simulink model "COMPONENT_MDL_Lag_QUAD_and_PEND_with_Ab"  (R2020b)
(part 8 of 12)

_Theta_pend))./2.0).*2.0+THE_Theta_D.*cos(THE_Psi).*sin(THE_Theta).*((Lz_pend.*THE_Psi_pend_D.*cos(THE_Theta_pend).*sin(THE_Psi_pend))./2.0+(Lz_pend.*THE_Theta_pend_D.*cos(THE_Psi_pend).*sin(THE_Theta_pend))./2.0).*2.0+Lz_pend.*THE_Psi_D.*cos(THE_Psi).*cos(THE_Theta).*(-THE_Psi_pend_D.*cos(THE_Phi_pend).*cos(THE_Psi_pend)+THE_Phi_pend_D.*sin(THE_Phi_pend).*sin(THE_Psi_pend)-THE_Psi_pend_D.*sin(THE_Phi_pend).*sin(THE_Psi_pend).*sin(THE_Theta_pend)+THE_Phi_pend_D.*cos(THE_Phi_pend).*cos(THE_Psi_pend).*sin(THE_Theta_pend)+THE_Theta_pend_D.*cos(THE_Psi_pend).*cos(THE_Theta_pend).*sin(THE_Phi_pend))-Lz_pend.*THE_Theta_D.*sin(THE_Psi).*sin(THE_Theta).*(-THE_Psi_pend_D.*cos(THE_Phi_pend).*cos(THE_Psi_pend)+THE_Phi_pend_D.*sin(THE_Phi_pend).*sin(THE_Psi_pend)-THE_Psi_pend_D.*sin(THE_Phi_pend).*sin(THE_Psi_pend).*sin(THE_Theta_pend)+THE_Phi_pend_D.*cos(THE_Phi_pend).*cos(THE_Psi_pend).*sin(THE_Theta_pend)+THE_Theta_pend_D.*cos(THE_Psi_pend).*cos(THE_Theta_pend).*sin(THE_Phi_pend))+THE_Psi_D.*THE_Theta_D.*sin(THE_Psi).*sin(THE_Theta).*(Tv_Z_pend+(Lz_pend.*cos(THE_Psi_pend).*cos(THE_Theta_pend))./2.0).*2.0+(Lz_pend.*THE_Psi_D.^2.*cos(THE_Theta).*sin(THE_Psi).*(cos(THE_Phi_pend).*sin(THE_Psi_pend)-cos(THE_Psi_pend).*sin(THE_Phi_pend).*sin(THE_Theta_pend)))./2.0+(Lz_pend.*THE_Theta_D.^2.*cos(THE_Theta).*sin(THE_Psi).*(cos(THE_Phi_pend).*sin(THE_Psi_pend)-cos(THE_Psi_pend).*sin(THE_Phi_pend).*sin(THE_Theta_pend)))./2.0+Lz_pend.*THE_Psi_D.*THE_Theta_D.*cos(THE_Psi).*sin(THE_Theta).*(cos(THE_Phi_pend).*sin(THE_Psi_pend)-cos(THE_Psi_pend).*sin(THE_Phi_pend).*sin(THE_Theta_pend)))+m_pend.*((Lz_pend.*cos(THE_Theta).*(sin(THE_Phi_pend).*sin(THE_Psi_pend)+cos(THE_Phi_pend).*cos(THE_Psi_pend).*sin(THE_Theta_pend)))./2.0+cos(THE_Psi).*sin(THE_Theta).*(Tv_Z_pend+(Lz_pend.*cos(THE_Psi_pend).*cos(THE_Theta_pend))./2.0)-(Lz_pend.*sin(THE_Psi).*sin(THE_Theta).*(cos(THE_Phi_pend).*sin(THE_Psi_pend)-cos(THE_Psi_pend).*sin(THE_Phi_pend).*sin(THE_Theta_pend)))./2.0).*((Lz_pend.*sin(THE_Theta).*(THE_Phi_pend_D.^2.*sin(THE_Phi_pend).*sin(THE_Psi_pend)+THE_Psi_pend_D.^2.*sin(THE_Phi_pend).*sin(THE_Psi_pend)+THE_Phi_pend_D.^2.*cos(THE_Phi_pend).*cos(THE_Psi_pend).*sin(THE_Theta_pend)+THE_Psi_pend_D.^2.*cos(THE_Phi_pend).*cos(THE_Psi_pend).*sin(THE_Theta_pend)+THE_Theta_pend_D.^2.*cos(THE_Phi_pend).*cos(THE_Psi_pend).*sin(THE_Theta_pend)-THE_Phi_pend_D.*THE_Psi_pend_D.*cos(THE_Phi_pend).*cos(THE_Psi_pend).*2.0+THE_Phi_pend_D.*THE_Theta_pend_D.*cos(THE_Psi_pend).*cos(THE_Theta_pend).*sin(THE_Phi_pend).*2.0+THE_Psi_pend_D.*THE_Theta_pend_D.*cos(THE_Phi_pend).*cos(THE_Theta_pend).*sin(THE_Psi_pend).*2.0-THE_Phi_pend_D.*THE_Psi_pend_D.*sin(THE_Phi_pend).*sin(THE_Psi_pend).*sin(THE_Theta_pend).*2.0))./4.0-(cos(THE_Psi).*cos(THE_Theta).*((Lz_pend.*THE_Psi_pend_D.^2.*cos(THE_Psi_pend).*cos(THE_Theta_pend))./2.0+(Lz_pend.*THE_Theta_pend_D.^2.*cos(THE_Psi_pend).*cos(THE_Theta_pend))./2.0-Lz_pend.*THE_Psi_pend_D.*THE_Theta_pend_D.*sin(THE_Psi_pend).*sin(THE_Theta_pend)))./2.0+(Lz_pend.*THE_Theta_D.^2.*sin(THE_Theta).*(sin(THE_Phi_pend).*sin(THE_Psi_pend)+cos(THE_Phi_pend).*cos(THE_Psi_pend).*sin(THE_Theta_pend)))./4.0-(Lz_pend.*cos(THE_Theta).*sin(THE_Psi).*(-THE_Phi_pend_D.^2.*cos(THE_Phi_pend).*sin(THE_Psi_pend)-THE_Psi_pend_D.^2.*cos(THE_Phi_pend).*sin(THE_Psi_pend)+THE_Phi_pend_D.^2.*cos(THE_Psi_pend).*sin(THE_Phi_pend).*sin(THE_Theta_pend)+THE_Psi_pend_D.^2.*cos(THE_Psi_pend).*sin(THE_Phi_pend).*sin(THE_Theta_pend)+THE_Theta_pend_D.^2.*cos(THE_Psi_pend).*sin(THE_Phi_pend).*sin(THE_Theta_pend)-THE_Phi_pend_D.*THE_Psi_pend_D.*cos(THE_Psi_pend).*sin(THE_Phi_pend).*2.0-THE_Phi_pend_D.*THE_Theta_pend_D.*cos(THE_Phi_pend).*cos(THE_Psi_pend).*cos(THE_Theta_pend).*2.0+THE_Phi_pend_D.*THE_Psi_pend_D.*cos(THE_Phi_pend).*sin(THE_Psi_pend).*sin(THE_Theta_pend).*2.0+THE_Psi_pend_D.*THE_Theta_pend_D.*cos(THE_Theta_pend).*sin(THE_Phi_pend).*sin(THE_Psi_pend).*2.0))./4.0-(Lz_pend.*THE_Theta_D.*cos(THE_Theta).*(THE_Phi_pend_D.*cos(THE_Phi_pend).*sin(THE_Psi_pend)+THE_Psi_pend_D.*cos(THE_Psi_pend).*sin(THE_Phi_pend)+THE_Theta_pend_D.*cos(THE_Phi_pend).*cos(THE_Psi_pend).*cos(THE_Theta_pend)-THE_Phi_pend_D.*cos(THE_Psi_pend).*sin(THE_Phi_pend).*sin(THE_Theta_pend)-THE_Psi_pend_D.*cos(THE_Phi_pend).*sin(THE_Psi_pend).*sin(THE_Theta_pend)))./2.0-(THE_Psi_D.^2.*cos(THE_Psi).*cos(THE_Theta).*(Tv_Z_pend+(Lz_pend.*cos(THE_Psi_pend).*cos(THE_Theta_pend))./2.0))./2.0-(THE_Theta_D.^2.*cos(THE_Psi).*cos(THE_Theta).*(Tv_Z_pend+(Lz_pend.*cos(THE_Psi_pend).*cos(THE_Theta_pend))./2.0))./2.0+THE_Psi_D.*cos(THE_Theta).*sin(THE_Psi).*((Lz_pend.*THE_Psi_pend_D.*cos(THE_Theta_pend).*sin(THE_Psi_pend))./2.0+(Lz_pend.*THE_Theta_pend_D.*cos(THE_Psi_pend).*sin(THE_Theta_pend))./2.0)+THE_Theta_D.*cos(THE_Psi).*sin(THE_Theta).*((Lz_pend.*THE_Psi_pend_D.*cos(THE_Theta_pend).*sin(THE_Psi_pend))./2.0+(Lz_pend.*THE_Theta_pend_D.*cos(THE_Psi_pend).*sin(THE_Theta_pend))./2.0)+(Lz_pend.*THE_Psi_D.*cos(THE_Psi).*cos(THE_Theta).*(-THE_Psi_pend_D.*cos(THE_Phi_pend).*cos(THE_Psi_pend)+THE_Phi_pend_D.*sin(THE_Phi_pend).*sin(THE_Psi_pend)-THE_Psi_pend_D.*sin(THE_Phi_pend).*sin(THE_Psi_pend).*sin(THE_Theta_pend)+THE_Phi_pend_D.*cos(THE_Phi_pend).*cos(THE_Psi_pend).*sin(THE_Theta_pend)+THE_Theta_pend_D.*cos(THE_Psi_pend).*cos(THE_Theta_pend).*sin(THE_Phi_pend)))./2.0-(Lz_pend.*THE_Theta_D.*sin(THE_Psi).*sin(THE_Theta).*(-THE_Psi_pend_D.*cos(THE_Phi_pend).*cos(THE_Psi_pend)+THE_Phi_pend_D.*sin(THE_Phi_pend).*sin(THE_Psi_pend)-THE_Psi_pend_D.*sin(THE_Phi_pend).*sin(THE_Psi_pend).*sin(THE_Theta_pend)+THE_Phi_pend_D.*cos(THE_Phi_pend).*cos(THE_Psi_pend).*sin(THE_Theta_pend)+THE_Theta_pend_D.*cos(THE_Psi_pend).*cos(THE_Theta_pend).*sin(THE_Phi_pend)))./2.0+THE_Psi_D.*THE_Theta_D.*sin(THE_Psi).*sin(THE_Theta).*(Tv_Z_pend+(Lz_pend.*cos(THE_Psi_pend).*cos(THE_Theta_pend))./2.0)+(Lz_pend.*THE_Psi_D.^2.*cos(THE_Theta).*sin(THE_Psi).*(cos(THE_Phi_pend).*sin(THE_Psi_pend)-cos(THE_Psi_pend).*sin(THE_Phi_pend).*sin(THE_Theta_pend)))./4.0+(Lz_pend.*THE_Theta_D.^2.*cos(THE_Theta).*sin(THE_Psi).*(cos(THE_Phi_pend).*sin(THE_Psi_pend)-cos(THE_Psi_pend).*sin(THE_Phi_pend).*sin(THE_Theta_pend)))./4.0+(Lz_pend.*THE_Psi_D.*THE_Theta_D.*cos(THE_Psi).*sin(THE_Theta).*(cos(THE_Phi_pend).*sin(THE_Psi_pend)-cos(THE_Psi_pend).*sin(THE_Phi_pend).*sin(THE_Theta_pend)))./2.0)-mprop.*(THE_Y_D-(cg_to_mot_L.*(THE_Theta_D.*sin(THE_Psi)-THE_Phi_D.*cos(THE_Psi).*cos(THE_Theta))+cg_to_mot_H.*(THE_Psi_D-THE_Phi_D.*sin(THE_Theta))).*(cos(THE_Phi).*cos(THE_Psi)+sin(THE_Phi).*sin(THE_Psi).*sin(THE_Theta))+cg_to_mot_L.*(cos(THE_Phi).*sin(THE_Psi)-cos(THE_Psi).*sin(THE_Phi).*sin(THE_Theta)).*(THE_Theta_D.*cos(THE_Psi)+THE_Phi_D.*cos(THE_Theta).*sin(THE_Psi))+cg_to_mot_H.*cos(THE_Theta).*sin(THE_Phi).*(THE_Theta_D.*cos(THE_Psi)+THE_Phi_D.*cos(THE_Theta).*sin(THE_Psi))).*((THE_Phi_D.*cg_to_mot_H.*cos(THE_Theta)-THE_Phi_D.*cg_to_mot_L.*cos(THE_Psi).*sin(THE_Theta)).*(cos(THE_Phi).*cos(THE_Psi)+sin(THE_Phi).*sin(THE_Psi).*sin(THE_Theta)).*(-1.0./2.0)+(cg_to_mot_H.*sin(THE_Phi).*sin(THE_Theta).*(THE_Theta_D.*cos(THE_Psi)+THE_Phi_D.*cos(THE_Theta).*sin(THE_Psi)))./2.0+(cos(THE_Theta).*sin(THE_Phi).*sin(THE_Psi).*(cg_to_mot_L.*(THE_Theta_D.*sin(THE_Psi)-THE_Phi_D.*cos(THE_Psi).*cos(THE_Theta))+cg_to_mot_H.*(THE_Psi_D-THE_Phi_D.*sin(THE_Theta))))./2.0+(THE_Phi_D.*cg_to_mot_L.*sin(THE_Psi).*sin(THE_Theta).*(cos(THE_Phi).*sin(THE_Psi)-cos(THE_Psi).*sin(THE_Phi).*sin(THE_Theta)))./2.0+(cg_to_mot_L.*cos(THE_Psi).*cos(THE_Theta).*sin(THE_Phi).*(THE_Theta_D.*cos(THE_Psi)+THE_Phi_D.*cos(THE_Theta).*sin(THE_Psi)))./2.0+(THE_Phi_D.*cg_to_mot_H.*cos(THE_Theta).*sin(THE_Phi).*sin(THE_Psi).*sin(THE_Theta))./2.0)+mprop.*(THE_Y_D+(cg_to_mot_L.*(THE_Theta_D.*sin(THE_Psi)-THE_Phi_D.*cos(THE_Psi).*cos(THE_Theta))-cg_to_mot_H.*(THE_Psi_D-THE_Phi_D.*sin(THE_Theta))).*(cos(THE_Phi).*cos(THE_Psi)+sin(THE_Phi).*sin(THE_Psi).*sin(THE_Theta))-cg_to_mot_L.*(cos(THE_Phi).*sin(THE_Psi)-cos(THE_Psi).*sin(THE_Phi).*sin(THE_Theta)).*(THE_Theta_D.*cos(THE_Psi)+THE_Phi_D.*cos(THE_Theta).*sin(THE_Psi))+cg_to_mot_H.*cos(THE_Theta).*sin(THE_Phi).*(THE_Theta_D.*cos(THE_Psi)+THE_Phi_D.*cos(THE_Theta).*sin(THE_Psi))).*(((THE_Phi_D.*cg_to_mot_H.*cos(THE_Theta)+THE_Phi_D.*cg_to_mot_L.*cos(THE_Psi).*sin(THE_Theta)).*(cos(THE_Phi).*cos(THE_Psi)+sin(THE_Phi).*sin(THE_Psi).*sin(THE_Theta)))./2.0-(cg_to_mot_H.*sin(THE_Phi).*sin(THE_Theta).*(THE_Theta_D.*cos(THE_Psi)+THE_Phi_D.*cos(THE_Theta).*sin(THE_Psi)))./2.0+(cos(THE_Theta).*sin(THE_Phi).*sin(THE_Psi).*(cg_to_mot_L.*(THE_Theta_D.*sin(THE_Psi)-THE_Phi_D.*cos(THE_Psi).*cos(THE_Theta))-cg_to_mot_H.*(THE_Psi_D-THE_Phi_D.*sin(THE_Theta))))./2.0+(THE_Phi_D.*cg_to_mot_L.*sin(THE_Psi).*sin(THE_Theta).*(cos(THE_Phi).*sin(THE_Psi)-cos(THE_Psi).*sin(THE_Phi).*sin(THE_Theta)))./2.0+(cg_to_mot_L.*cos(THE_Psi).*cos(THE_Theta).*sin(THE_Phi).*(THE_Theta_D.*cos(THE_Psi)+THE_Phi_D.*cos(THE_Theta).*sin(THE_Psi)))./2.0-(THE_Phi_D.*cg_to_mot_H.*cos(THE_Theta).*sin(THE_Phi).*sin(THE_Psi).*sin(THE_Theta))./2.0)-mprop.*(THE_X_D./2.0+((cg_to_mot_L.*(THE_Theta_D.*sin(THE_Psi)-THE_Phi_D.*cos(THE_Psi).*cos(THE_Theta))+cg_to_mot_H.*(THE_Psi_D-THE_Phi_D.*sin(THE_Theta))).*(cos(THE_Psi).*sin(THE_Phi)-cos(THE_Phi).*sin(THE_Psi).*sin(THE_Theta)))./2.0-(cg_to_mot_L.*(sin(THE_Phi).*sin(THE_Psi)+cos(THE_Phi).*cos(THE_Psi).*sin(THE_Theta)).*(THE_Theta_D.*cos(THE_Psi)+THE_Phi_D.*cos(THE_Theta).*sin(THE_Psi)))./2.0+(cg_to_mot_H.*cos(THE_Phi).*cos(THE_Theta).*(THE_Theta_D.*cos(THE_Psi)+THE_Phi_D.*cos(THE_Theta).*sin(THE_Psi)))./2.0).*((THE_Phi_D.*cg_to_mot_H.*cos(THE_Theta)-THE_Phi_D.*cg_to_mot_L.*cos(THE_Psi).*sin(THE_Theta)).*(cos(THE_Psi).*sin(THE_Phi)-cos(THE_Phi).*sin(THE_Psi).*sin(THE_Theta))+cg_to_mot_H.*cos(THE_Phi).*sin(THE_Theta).*(THE_Theta_D.*cos(THE_Psi)+THE_Phi_D.*cos(THE_Theta).*sin(THE_Psi))+cos(THE_Phi).*cos(THE_Theta).*sin(THE_Psi).*(cg_to_mot_L.*(THE_Theta_D.*sin(THE_Psi)-THE_Phi_D.*cos(THE_Psi).*cos(THE_Theta))+cg_to_mot_H.*(THE_Psi_D-THE_Phi_D.*sin(THE_Theta)))-THE_Phi_D.*cg_to_mot_L.*sin(THE_Psi).*sin(THE_Theta).*(sin(THE_Phi).*sin(THE_Psi)+cos(THE_Phi).*cos(THE_Psi).*sin(THE_Theta))+cg_to_mot_L.*cos(THE_Phi).*cos(THE_Psi).*cos(THE_Theta).*(THE_Theta_D.*cos(THE_Psi)+THE_Phi_D.*cos(THE_Theta).*sin(THE_Psi))+THE_Phi_D.*cg_to_mot_H.*cos(THE_Phi).*cos(THE_Theta).*sin(THE_Psi).*sin(THE_Theta))-mprop.*(THE_X_D./2.0-((cg_to_mot_L.*(THE_Theta_D.*sin(THE_Psi)-THE_Phi_D.*cos(THE_Psi).*cos(THE_Theta))-cg_to_mot_H.*(THE_Psi_D-THE_Phi_D.*sin(THE_Theta))).*(cos(THE_Psi).*sin(THE_Phi)-cos(THE_Phi).*sin(THE_Psi).*sin(THE_Theta)))./2.0+(cg_to_mot_L.*(sin(THE_Phi).*sin(THE_Psi)+cos(THE_Phi).*cos(THE_Psi).*sin(THE_Theta)).*(THE_Theta_D.*cos(THE_Psi)+THE_Phi_D.*cos(THE_Theta).*sin(THE_Psi)))./2.0+(cg_to_mot_H.*cos(THE_Phi).*cos(THE_Theta).*(THE_Theta_D.*cos(THE_Psi)+THE_Phi_D.*cos(THE_Theta).*sin(THE_Psi)))./2.0).*((THE_Phi_D.*cg_to_mot_H.*cos(THE_Theta)+THE_Phi_D.*cg_to_mot_L.*cos(THE_Psi).*sin(THE_Theta)).*(cos(THE_Psi).*sin(THE_Phi)-cos(THE_Phi).*sin(THE_Psi).*sin(THE_Theta))+cg_to_mot_H.*cos(THE_Phi).*sin(THE_Theta).*(THE_Theta_D.*cos(THE_Psi)+THE_Phi_D.*cos(THE_Theta).*sin(THE_Psi))-cos(THE_Phi).*cos(THE_Theta).*sin(THE_Psi).*(cg_to_mot_L.*(THE_Theta_D.*sin(THE_Psi)-THE_Phi_D.*cos(THE_Psi).*cos(THE_Theta))-cg_to_mot_H.*(THE_Psi_D-THE_Phi_D.*sin(THE_Theta)))+THE_Phi_D.*cg_to_mot_L.*sin(THE_Psi).*sin(THE_Theta).*(sin(THE_Phi).*sin(THE_Psi)+cos(THE_Phi).*cos(THE_Psi).*sin(THE_Theta))-cg_to_mot_L.*cos(THE_Phi).*cos(THE_Psi).*cos(THE_Theta).*(THE_Theta_D.*cos(THE_Psi)+THE_Phi_D.*cos(THE_Theta).*sin(THE_Psi))+THE_Phi_D.*cg_to_mot_H.*cos(THE_Phi).*cos(THE_Theta).*sin(THE_Psi).*sin(THE_Theta))+mprop.*(cg_to_mot_L.*cos(THE_Psi).*(sin(THE_Phi).*sin(THE_Psi)+cos(THE_Phi).*cos(THE_Psi).*sin(THE_Theta)).*(-1.0./2.0)+(cg_to_mot_L.*sin(THE_Psi).*(cos(THE_Psi).*sin(THE_Phi)-cos(THE_Phi).*sin(THE_Psi).*sin(THE_Theta)))./2.0+(cg_to_mot_H.*cos(THE_Phi).*cos(THE_Psi).*cos(THE_Theta))./2.0).*((cg_to_mot_L.*(THE_Theta_D.*sin(THE_Psi)-THE_Phi_D.*cos(THE_Psi).*cos(THE_Theta))+cg_to_mot_H.*(THE_Psi_D-THE_Phi_D.*sin(THE_Theta))).*(-THE_Phi_D.*cos(THE_Phi).*cos(THE_Psi)+THE_Psi_D.*sin(THE_Phi).*sin(THE_Psi)-THE_Phi_D.*sin(THE_Phi).*sin(THE_Psi).*sin(THE_Theta)+THE_Psi_D.*cos(THE_Phi).*cos(THE_Psi).*sin(THE_Theta)+THE_Theta_D.*cos(THE_Phi).*cos(THE_Theta).*sin(THE_Psi))-(cg_to_mot_L.*(THE_Psi_D.*THE_Theta_D.*cos(THE_Psi)+THE_Phi_D.*THE_Psi_D.*cos(THE_Theta).*sin(THE_Psi)+THE_Phi_D.*THE_Theta_D.*cos(THE_Psi).*sin(THE_Theta))-THE_Phi_D.*THE_Theta_D.*cg_to_mot_H.*cos(THE_Theta)).*(cos(THE_Psi).*sin(THE_Phi)-cos(THE_Phi).*sin(THE_Psi).*sin(THE_Theta))+cg_to_mot_L.*(THE_Theta_D.*cos(THE_Psi)+THE_Phi_D.*cos(THE_Theta).*sin(THE_Psi)).*(THE_Phi_D.*cos(THE_Phi).*sin(THE_Psi)+THE_Psi_D.*cos(THE_Psi).*sin(THE_Phi)+THE_Theta_D.*cos(THE_Phi).*cos(THE_Psi).*cos(THE_Theta)-THE_Phi_D.*cos(THE_Psi).*sin(THE_Phi).*sin(THE_Theta)-THE_Psi_D.*cos(THE_Phi).*sin(THE_Psi).*sin(THE_Theta))-cg_to_mot_L.*(sin(THE_Phi).*sin(THE_Psi)+cos(THE_Phi).*cos(THE_Psi).*sin(THE_Theta)).*(THE_Psi_D.*THE_Theta_D.*sin(THE_Psi)-THE_Phi_D.*THE_Psi_D.*cos(THE_Psi).*cos(THE_Theta)+THE_Phi_D.*THE_Theta_D.*sin(THE_Psi).*sin(THE_Theta))+cg_to_mot_H.*cos(THE_Phi).*cos(THE_Theta).*(THE_Psi_D.*THE_Theta_D.*sin(THE_Psi)-THE_Phi_D.*THE_Psi_D.*cos(THE_Psi).*cos(THE_Theta)+THE_Phi_D.*THE_Theta_D.*sin(THE_Psi).*sin(THE_Theta))+THE_Phi_D.*cg_to_mot_H.*cos(THE_Theta).*sin(THE_Phi).*(THE_Theta_D.*cos(THE_Psi)+THE_Phi_D.*cos(THE_Theta).*sin(THE_Psi))+THE_Theta_D.*cg_to_mot_H.*cos(THE_Phi).*sin(THE_Theta).*(THE_Theta_D.*cos(THE_Psi)+THE_Phi_D.*cos(THE_Theta).*sin(THE_Psi)))+mprop.*((cg_to_mot_L.*cos(THE_Psi).*(sin(THE_Phi).*sin(THE_Psi)+cos(THE_Phi).*cos(THE_Psi).*sin(THE_Theta)))./2.0-(cg_to_mot_L.*sin(THE_Psi).*(cos(THE_Psi).*sin(THE_Phi)-cos(THE_Phi).*sin(THE_Psi).*sin(THE_Theta)))./2.0+(cg_to_mot_H.*cos(THE_Phi).*cos(THE_Psi).*cos(THE_Theta))./2.0).*(-(cg_to_mot_L.*(THE_Theta_D.*sin(THE_Psi)-THE_Phi_D.*cos(THE_Psi).*cos(THE_Theta))-cg_to_mot_H.*(THE_Psi_D-THE_Phi_D.*sin(THE_Theta))).*(-THE_Phi_D.*cos(THE_Phi).*cos(THE_Psi)+THE_Psi_D.*sin(THE_Phi).*sin(THE_Psi)-THE_Phi_D.*sin(THE_Phi).*sin(THE_Psi).*sin(THE_Theta)+THE_Psi_D.*cos(THE_Phi).*cos(THE_Psi).*sin(THE_Theta)+THE_Theta_D.*cos(THE_Phi).*cos(THE_Theta).*sin(THE_Psi))+(cg_to_mot_L.*(THE_Psi_D.*THE_Theta_D.*cos(THE_Psi)+THE_Phi_D.*THE_Psi_D.*cos(THE_Theta).*sin(THE_Psi)+THE_Phi_D.*THE_Theta_D.*cos(THE_Psi).*sin(THE_Theta))+THE_Phi_D.*THE_Theta_D.*cg_to_mot_H.*cos(THE_Theta)).*(cos(THE_Psi).*sin(THE_Phi)-cos(THE_Phi).*sin(THE_Psi).*sin(THE_Theta))-cg_to_mot_L.*(THE_Theta_D.*cos(THE_Psi)+THE_Phi_D.*cos(THE_Theta).*sin(THE_Psi)).*(THE_Phi_D.*cos(THE_Phi).*sin(THE_Psi)+THE_Psi_D.*cos(THE_Psi).*sin(THE_Phi)+THE_Theta_D.*cos(THE_Phi).*cos(THE_Psi).*cos(THE_Theta)-THE_Phi_D.*cos(THE_Psi).*sin(THE_Phi).*sin(THE_Theta)-THE_Psi_D.*cos(THE_Phi).*sin(THE_Psi).*sin(THE_Theta))+cg_to_mot_L.*(sin(THE_Phi).*sin(THE_Psi)+cos(THE_Phi).*cos(THE_Psi).*sin(THE_Theta)).*(THE_Psi_D.*THE_Theta_D.*sin(THE_Psi)-THE_Phi_D.*THE_Psi_D.*cos(THE_Psi).*cos(THE_Theta)+THE_Phi_D.*THE_Theta_D.*sin(THE_Psi).*sin(THE_Theta))+cg_to_mot_H.*cos(THE_Phi).*cos(THE_Theta).*(THE_Psi_D.*THE_Theta_D.*sin(THE_Psi)-THE_Phi_D.*THE_Psi_D.*cos(THE_Psi).*cos(THE_Theta)+THE_Phi_D.*THE_Theta_D.*sin(THE_Psi).*sin(THE_Theta))+THE_Phi_D.*cg_to_mot_H.*cos(THE_Theta).*sin(THE_Phi).*(THE_Theta_D.*cos(THE_Psi)+THE_Phi_D.*cos(THE_Theta).*sin(THE_Psi))+THE_Theta_D.*cg_to_mot_H.*cos(THE_Phi).*sin(THE_Theta).*(THE_Theta_D.*cos(THE_Psi)+THE_Phi_D.*cos(THE_Theta).*sin(THE_Psi)))+mprop.*(cg_to_mot_L.*cos(THE_Psi).*(sin(THE_Phi).*sin(THE_Psi)+cos(THE_Phi).*cos(THE_Psi).*sin(THE_Theta))-cg_to_mot_L.*sin(THE_Psi).*(cos(THE_Psi).*sin(THE_Phi)-cos(THE_Phi).*sin(THE_Psi).*sin(THE_Theta))+cg_to_mot_H.*cos(THE_Phi).*cos(THE_Psi).*cos(THE_Theta)).*((cg_to_mot_L.*(THE_Theta_D.*sin(THE_Psi)-THE_Phi_D.*cos(THE_Psi).*cos(THE_Theta))-cg_to_mot_H.*(THE_Psi_D-THE_Phi_D.*sin(THE_Theta))).*(-THE_Phi_D.*cos(THE_Phi).*cos(THE_Psi)+THE_Psi_D.*sin(THE_Phi).*sin(THE_Psi)-THE_Phi_D.*sin(THE_Phi).*sin(THE_Psi).*sin(THE_Theta)+THE_Psi_D.*cos(THE_Phi).*cos(THE_Psi).*sin(THE_Theta)+THE_Theta_D.*cos(THE_Phi).*cos(THE_Theta).*sin(THE_Psi)).*(-1.0./2.0)+((cg_to_mot_L.*(THE_Psi_D.*THE_Theta_D.*cos(THE_Psi)+THE_Phi_D.*THE_Psi_D.*cos(THE_Theta).*sin(THE_Psi)+THE_Phi_D.*THE_Theta_D.*cos(THE_Psi).*sin(THE_Theta))+THE_Phi_D.*THE_Theta_D.*cg_to_mot_H.*cos(THE_Theta)).*(cos(THE_Psi).*sin(THE_Phi)-cos(THE_Phi).*sin(THE_Psi).*sin(THE_Theta)))./2.0-(cg_to_mot_L.*(THE_Theta_D.*cos(THE_Psi)+THE_Phi_D.*cos(THE_Theta).*sin(THE_Psi)).*(THE_Phi_D.*cos(THE_Phi).*sin(THE_Psi)+THE_Psi_D.*cos(THE_Psi).*sin(THE_Phi)+THE_Theta_D.*cos(THE_Phi).*cos(THE_Psi).*cos(THE_Theta)-THE_Phi_D.*cos(THE_Psi).*sin(THE_Phi).*sin(THE_Theta)-THE_Psi_D.*cos(THE_Phi).*sin(THE_Psi).*sin(THE_Theta)))./2.0+(cg_to_mot_L.*(sin(THE_Phi).*sin(THE_Psi)+cos(THE_Phi).*cos(THE_Psi).*sin(THE_Theta)).*(THE_Psi_D.*THE_Theta_D.*sin(THE_Psi)-THE_Phi_D.*THE_Psi_D.*cos(THE_Psi).*cos(THE_Theta)+THE_Phi_D.*THE_Theta_D.*sin(THE_Psi).*sin(THE_Theta)))./2.0+(cg_to_mot_H.*cos(THE_Phi).*cos(THE_Theta).*(THE_Psi_D.*THE_Theta_D.*sin(THE_Psi)-THE_Phi_D.*THE_Psi_D.*cos(THE_Psi).*cos(THE_Theta)+THE_Phi_D.*THE_Theta_D.*sin(THE_Psi).*sin(THE_Theta)))./2.0+(THE_Phi_D.*cg_to_mot_H.*cos(THE_Theta).*sin(THE_Phi).*(THE_Theta_D.*cos(THE_Psi)+THE_Phi_D.*cos(THE_Theta).*sin(THE_Psi)))./2.0+(THE_Theta_D.*cg_to_mot_H.*cos(THE_Phi).*sin(THE_Theta).*(THE_Theta_D.*cos(THE_Psi)+THE_Phi_D.*cos(THE_Theta).*sin(THE_Psi)))./2.0)+mprop.*(-cg_to_mot_L.*cos(THE_Psi).*(sin(THE_Phi).*sin(THE_Psi)+cos(THE_Phi).*cos(THE_Psi).*sin(THE_Theta))+cg_to_mot_L.*sin(THE_Psi).*(cos(THE_Psi).*sin(THE_Phi)-cos(THE_Phi).*sin(THE_Psi).*sin(THE_Theta))+cg_to_mot_H.*cos(THE_Phi).*cos(THE_Psi).*cos(THE_Theta)).*(((cg_to_mot_L.*(THE_Theta_D.*sin(THE_Psi)-THE_Phi_D.*cos(THE_Psi).*cos(THE_Theta))+cg_to_mot_H.*(THE_Psi_D-THE_Phi_D.*sin(THE_Theta))).*(-THE_Phi_D.*cos(THE_Phi).*cos(THE_Psi)+THE_Psi_D.*sin(THE_Phi).*sin(THE_Psi)-THE_Phi_D.*sin(THE_Phi).*sin(THE_Psi).*sin(THE_Theta)+THE_Psi_D.*cos(THE_Phi).*cos(THE_Psi).*sin(THE_Theta)+THE_Theta_D.*cos(THE_Phi).*cos(THE_Theta).*sin(THE_Psi)))./2.0-((cg_to_mot_L.*(THE_Psi_D.*THE_Theta_D.*cos(THE_Psi)+THE_Phi_D.*THE_Psi_D.*cos(THE_Theta).*sin(THE_Psi)+THE_Phi_D.*THE_Theta_D.*cos(THE_Psi).*sin(THE_Theta))-THE_Phi_D.*THE_Theta_D.*cg_to_mot_H.*cos(THE_Theta)).*(cos(THE_Psi).*sin(THE_Phi)-cos(THE_Phi).*sin(THE_Psi).*sin(THE_Theta)))./2.0+(cg_to_mot_L.*(THE_Theta_D.*cos(THE_Psi)+THE_Phi_D.*cos(THE_Theta).*sin(THE_Psi)).*(THE_Phi_D.*cos(THE_Phi).*sin(THE_Psi)+THE_Psi_D.*cos(THE_Psi).*sin(THE_Phi)+THE_Theta_D.*cos(THE_Phi).*cos(THE_Psi).*cos(THE_Theta)-THE_Phi_D.*cos(THE_Psi).*sin(THE_Phi).*sin(THE_Theta)-THE_Psi_D.*cos(THE_Phi).*sin(THE_Psi).*sin(THE_Theta)))./2.0-(cg_to_mot_L.*(sin(THE_Phi).*sin(THE_Psi)+cos(THE_Phi).*cos(THE_Psi).*sin(THE_Theta)).*(THE_Psi_D.*THE_Theta_D.*sin(THE_Psi)-THE_Phi_D.*THE_Psi_D.*cos(THE_Psi).*cos(THE_Theta)+THE_Phi_D.*THE_Theta_D.*sin(THE_Psi).*sin(THE_Theta)))./2.0+(cg_to_mot_H.*cos(THE_Phi).*cos(THE_Theta).*(THE_Psi_D.*THE_Theta_D.*sin(THE_Psi)-THE_Phi_D.*THE_Psi_D.*cos(THE_Psi).*cos(THE_Theta)+THE_Phi_D.*THE_Theta_D.*sin(THE_Psi).*sin(THE_Theta)))./2.0+(THE_Phi_D.*cg_to_mot_H.*cos(THE_Theta).*sin(THE_Phi).*(THE_Theta_D.*cos(THE_Psi)+THE_Phi_D.*cos(THE_Theta).*sin(THE_Psi)))./2.0+(THE_Theta_D.*cg_to_mot_H.*cos(THE_Phi).*sin(THE_Theta).*(THE_Theta_D.*cos(THE_Psi)+THE_Phi_D.*cos(THE_Theta).*sin(THE_Psi)))./2.0)+mprop.*(THE_Y_D-(cg_to_mot_L.*(THE_Theta_D.*sin(THE_Psi)-THE_Phi_D.*cos(THE_Psi).*cos(THE_Theta))+cg_to_mot_H.*(THE_Psi_D-THE_Phi_D.*sin(THE_Theta))).*(cos(THE_Phi).*cos(THE_Psi)+sin(THE_Phi).*sin(THE_Psi).*sin(THE_Theta))+cg_to_mot_L.*(cos(THE_Phi).*sin(THE_Psi)-cos(THE_Psi).*sin(THE_Phi).*sin(THE_Theta)).*(THE_Theta_D.*cos(THE_Psi)+THE_Phi_D.*cos(THE_Theta).*sin(THE_Psi))+cg_to_mot_H.*cos(THE_Theta).*sin(THE_Phi).*(THE_Theta_D.*cos(THE_Psi)+THE_Phi_D.*cos(THE_Theta).*sin(THE_Psi))).*((cg_to_mot_L.*cos(THE_Psi).*(-THE_Psi_D.*cos(THE_Phi).*cos(THE_Psi)+THE_Phi_D.*sin(THE_Phi).*sin(THE_Psi)-THE_Psi_D.*sin(THE_Phi).*sin(THE_Psi).*sin(THE_Theta)+THE_Phi_D.*cos(THE_Phi).*cos(THE_Psi).*sin(THE_Theta)+THE_Theta_D.*cos(THE_Psi).*cos(THE_Theta).*sin(THE_Phi)))./2.0+(cg_to_mot_L.*sin(THE_Psi).*(-THE_Phi_D.*cos(THE_Psi).*sin(THE_Phi)-THE_Psi_D.*cos(THE_Phi).*sin(THE_Psi)+THE_Phi_D.*cos(THE_Phi).*sin(THE_Psi).*sin(THE_Theta)+THE_Psi_D.*cos(THE_Psi).*sin(THE_Phi).*sin(THE_Theta)+THE_Theta_D.*cos(THE_Theta).*sin(THE_Phi).*sin(THE_Psi)))./2.0+(THE_Psi_D.*cg_to_mot_L.*cos(THE_Psi).*(cos(THE_Phi).*cos(THE_Psi)+sin(THE_Phi).*sin(THE_Psi).*sin(THE_Theta)))./2.0+(THE_Psi_D.*cg_to_mot_L.*sin(THE_Psi).*(cos(THE_Phi).*sin(THE_Psi)-cos(THE_Psi).*sin(THE_Phi).*sin(THE_Theta)))./2.0-(THE_Phi_D.*cg_to_mot_H.*cos(THE_Phi).*cos(THE_Psi).*cos(THE_Theta))./2.0+(THE_Psi_D.*cg_to_mot_H.*cos(THE_Theta).*sin(THE_Phi).*sin(THE_Psi))./2.0+(THE_Theta_D.*cg_to_mot_H.*cos(THE_Psi).*sin(THE_Phi).*sin(THE_Theta))./2.0)-mprop.*(THE_Y_D+(cg_to_mot_L.*(THE_Theta_D.*sin(THE_Psi)-THE_Phi_D.*cos(THE_Psi).*cos(THE_Theta))-cg_to_mot_H.*(THE_Psi_D-THE_Phi_D.*sin(THE_Theta))).*(cos(THE_Phi).*cos(THE_Psi)+sin(THE_Phi).*sin(THE_Psi).*sin(THE_Theta))-cg_to_mot_L.*(cos(THE_Phi).*sin(THE_Psi)-cos(THE_Psi).*sin(THE_Phi).*sin(THE_Theta)).*(THE_Theta_D.*cos(THE_Psi)+THE_Phi_D.*cos(THE_Theta).*sin(THE_Psi))+cg_to_mot_H.*cos(THE_Theta).*sin(THE_Phi).*(THE_Theta_D.*cos(THE_Psi)+THE_Phi_D.*cos(THE_Theta).*sin(THE_Psi))).*((cg_to_mot_L.*cos(THE_Psi).*(-THE_Psi_D.*cos(THE_Phi).*cos(THE_Psi)+THE_Phi_D.*sin(THE_Phi).*sin(THE_Psi)-THE_Psi_D.*sin(THE_Phi).*sin(THE_Psi).*sin(THE_Theta)+THE_Phi_D.*cos(THE_Phi).*cos(THE_Psi).*sin(THE_Theta)+THE_Theta_D.*cos(THE_Psi).*cos(THE_Theta).*sin(THE_Phi)))./2.0+(cg_to_mot_L.*sin(THE_Psi).*(-THE_Phi_D.*cos(THE_Psi).*sin(THE_Phi)-THE_Psi_D.*cos(THE_Phi).*sin(THE_Psi)+THE_Phi_D.*cos(THE_Phi).*sin(THE_Psi).*sin(THE_Theta)+THE_Psi_D.*cos(THE_Psi).*sin(THE_Phi).*sin(THE_Theta)+THE_Theta_D.*cos(THE_Theta).*sin(THE_Phi).*sin(THE_Psi)))./2.0+(THE_Psi_D.*cg_to_mot_L.*cos(THE_Psi).*(cos(THE_Phi).*cos(THE_Psi)+sin(THE_Phi).*sin(THE_Psi).*sin(THE_Theta)))./2.0+(THE_Psi_D.*cg_to_mot_L.*sin(THE_Psi).*(cos(THE_Phi).*sin(THE_Psi)-cos(THE_Psi).*sin(THE_Phi).*sin(THE_Theta)))./2.0+(THE_Phi_D.*cg_to_mot_H.*cos(THE_Phi).*cos(THE_Psi).*cos(THE_Theta))./2.0-(THE_Psi_D.*cg_to_mot_H.*cos(THE_Theta).*sin(THE_Phi).*sin(THE_Psi))./2.0-(THE_Theta_D.*cg_to_mot_H.*cos(THE_Psi).*sin(THE_Phi).*sin(THE_Theta))./2.0)-m_pend.*(Ly_pend.^2./1.2e+1+Lz_pend.^2./1.2e+1).*(THE_Psi_pend_D+sin(THE_Theta_pend).*(THE_Theta_D.*sin(THE_Psi)-THE_Phi_D.*cos(THE_Psi).*cos(THE_Theta))-THE_Phi_pend_D.*sin(THE_Theta_pend)+cos(THE_Theta_pend).*sin(THE_Phi_pend).*(THE_Theta_D.*cos(THE_Psi)+THE_Phi_D.*cos(THE_Theta).*sin(THE_Psi))+cos(THE_Phi_pend).*cos(THE_Theta_pend).*(THE_Psi_D-THE_Phi_D.*sin(THE_Theta))).*((THE_Psi_D.*cos(THE_Psi).*sin(THE_Theta_pend))./2.0+(THE_Theta_pend_D.*cos(THE_Theta_pend).*sin(THE_Psi))./2.0+(THE_Phi_pend_D.*cos(THE_Psi).*cos(THE_Phi_pend).*cos(THE_Theta_pend))./2.0-(THE_Psi_D.*cos(THE_Theta_pend).*sin(THE_Psi).*sin(THE_Phi_pend))./2.0-(THE_Theta_pend_D.*cos(THE_Psi).*sin(THE_Phi_pend).*sin(THE_Theta_pend))./2.0)+m_pend.*(Lx_pend.^2./1.2e+1+Ly_pend.^2./1.2e+1).*(cos(THE_Psi).*(-THE_Psi_pend_D.*cos(THE_Phi_pend).*cos(THE_Psi_pend)+THE_Phi_pend_D.*sin(THE_Phi_pend).*sin(THE_Psi_pend)-THE_Psi_pend_D.*sin(THE_Phi_pend).*sin(THE_Psi_pend).*sin(THE_Theta_pend)+THE_Phi_pend_D.*cos(THE_Phi_pend).*cos(THE_Psi_pend).*sin(THE_Theta_pend)+THE_Theta_pend_D.*cos(THE_Psi_pend).*cos(THE_Theta_pend).*sin(THE_Phi_pend))+THE_Psi_D.*sin(THE_Psi).*(cos(THE_Phi_pend).*sin(THE_Psi_pend)-cos(THE_Psi_pend).*sin(THE_Phi_pend).*sin(THE_Theta_pend))-THE_Psi_D.*cos(THE_Psi).*cos(THE_Psi_pend).*cos(THE_Theta_pend)+THE_Psi_pend_D.*cos(THE_Theta_pend).*sin(THE_Psi).*sin(THE_Psi_pend)+THE_Theta_pend_D.*cos(THE_Psi_pend).*sin(THE_Psi).*sin(THE_Theta_pend)).*(((cos(THE_Phi_pend).*sin(THE_Psi_pend)-cos(THE_Psi_pend).*sin(THE_Phi_pend).*sin(THE_Theta_pend)).*(THE_Theta_D.*cos(THE_Psi)+THE_Phi_D.*cos(THE_Theta).*sin(THE_Psi)))./2.0-((THE_Psi_D-THE_Phi_D.*sin(THE_Theta)).*(sin(THE_Phi_pend).*sin(THE_Psi_pend)+cos(THE_Phi_pend).*cos(THE_Psi_pend).*sin(THE_Theta_pend)))./2.0+(THE_Theta_pend_D.*sin(THE_Psi_pend))./2.0-(THE_Phi_pend_D.*cos(THE_Psi_pend).*cos(THE_Theta_pend))./2.0+(cos(THE_Psi_pend).*cos(THE_Theta_pend).*(THE_Theta_D.*sin(THE_Psi)-THE_Phi_D.*cos(THE_Psi).*cos(THE_Theta)))./2.0)+m_pend.*(Lx_pend.^2./1.2e+1+Ly_pend.^2./1.2e+1).*((cos(THE_Psi).*(-THE_Psi_pend_D.*cos(THE_Phi_pend).*cos(THE_Psi_pend)+THE_Phi_pend_D.*sin(THE_Phi_pend).*sin(THE_Psi_pend)-THE_Psi_pend_D.*sin(THE_Phi_pend).*sin(THE_Psi_pend).*sin(THE_Theta_pend)+THE_Phi_pend_D.*cos(THE_Phi_pend).*cos(THE_Psi_pend).*sin(THE_Theta_pend)+THE_Theta_pend_D.*cos(THE_Psi_pend).*cos(THE_Theta_pend).*sin(THE_Phi_pend)))./2.0+(THE_Psi_D.*sin(THE_Psi).*(cos(THE_Phi_pend).*sin(THE_Psi_pend)-cos(THE_Psi_pend).*sin(THE_Phi_pend).*sin(THE_Theta_pend)))./2.0-(THE_Psi_D.*cos(THE_Psi).*cos(THE_Psi_pend).*cos(THE_Theta_pend))./2.0+(THE_Psi_pend_D.*cos(THE_Theta_pend).*sin(THE_Psi).*sin(THE_Psi_pend))./2.0+(THE_Theta_pend_D.*cos(THE_Psi_pend).*sin(THE_Psi).*sin(THE_Theta_pend))./2.0).*((cos(THE_Phi_pend).*sin(THE_Psi_pend)-cos(THE_Psi_pend).*sin(THE_Phi_pend).*sin(THE_Theta_pend)).*(THE_Theta_D.*cos(THE_Psi)+THE_Phi_D.*cos(THE_Theta).*sin(THE_Psi))-(THE_Psi_D-THE_Phi_D.*sin(THE_Theta)).*(sin(THE_Phi_pend).*sin(THE_Psi_pend)+cos(THE_Phi_pend).*cos(THE_Psi_pend).*sin(THE_Theta_pend))+THE_Theta_pend_D.*sin(THE_Psi_pend)-THE_Phi_pend_D.*cos(THE_Psi_pend).*cos(THE_Theta_pend)+cos(THE_Psi_pend).*cos(THE_Theta_pend).*(THE_Theta_D.*sin(THE_Psi)-THE_Phi_D.*cos(THE_Psi).*cos(THE_Theta)))+m_pend.*(Lx_pend.^2./1.2e+1+Ly_pend.^2./1.2e+1).*((cos(THE_Psi).*(cos(THE_Phi_pend).*sin(THE_Psi_pend)-cos(THE_Psi_pend).*sin(THE_Phi_pend).*sin(THE_Theta_pend)))./2.0+(cos(THE_Psi_pend).*cos(THE_Theta_pend).*sin(THE_Psi))./2.0).*((THE_Theta_D.*cos(THE_Psi)+THE_Phi_D.*cos(THE_Theta).*sin(THE_Psi)).*(-THE_Psi_pend_D.*cos(THE_Phi_pend).*cos(THE_Psi_pend)+THE_Phi_pend_D.*sin(THE_Phi_pend).*sin(THE_Psi_pend)-THE_Psi_pend_D.*sin(THE_Phi_pend).*sin(THE_Psi_pend).*sin(THE_Theta_pend)+THE_Phi_pend_D.*cos(THE_Phi_pend).*cos(THE_Psi_pend).*sin(THE_Theta_pend)+THE_Theta_pend_D.*cos(THE_Psi_pend).*cos(THE_Theta_pend).*sin(THE_Phi_pend))+(THE_Psi_D-THE_Phi_D.*sin(THE_Theta)).*(THE_Phi_pend_D.*cos(THE_Phi_pend).*sin(THE_Psi_pend)+THE_Psi_pend_D.*cos(THE_Psi_pend).*sin(THE_Phi_pend)+THE_Theta_pend_D.*cos(THE_Phi_pend).*cos(THE_Psi_pend).*cos(THE_Theta_pend)-THE_Phi_pend_D.*cos(THE_Psi_pend).*sin(THE_Phi_pend).*sin(THE_Theta_pend)-THE_Psi_pend_D.*cos(THE_Phi_pend).*sin(THE_Psi_pend).*sin(THE_Theta_pend))+(cos(THE_Phi_pend).*sin(THE_Psi_pend)-cos(THE_Psi_pend).*sin(THE_Phi_pend).*sin(THE_Theta_pend)).*(THE_Psi_D.*THE_Theta_D.*sin(THE_Psi)-THE_Phi_D.*THE_Psi_D.*cos(THE_Psi).*cos(THE_Theta)+THE_Phi_D.*THE_Theta_D.*sin(THE_Psi).*sin(THE_Theta))-THE_Psi_pend_D.*THE_Theta_pend_D.*cos(THE_Psi_pend)-cos(THE_Psi_pend).*cos(THE_Theta_pend).*(THE_Psi_D.*THE_Theta_D.*cos(THE_Psi)+THE_Phi_D.*THE_Psi_D.*cos(THE_Theta).*sin(THE_Psi)+THE_Phi_D.*THE_Theta_D.*cos(THE_Psi).*sin(THE_Theta))+THE_Psi_pend_D.*cos(THE_Theta_pend).*sin(THE_Psi_pend).*(THE_Theta_D.*sin(THE_Psi)-THE_Phi_D.*cos(THE_Psi).*cos(THE_Theta))+THE_Theta_pend_D.*cos(THE_Psi_pend).*sin(THE_Theta_pend).*(THE_Theta_D.*sin(THE_Psi)-THE_Phi_D.*cos(THE_Psi).*cos(THE_Theta))-THE_Phi_pend_D.*THE_Psi_pend_D.*cos(THE_Theta_pend).*sin(THE_Psi_pend)-THE_Phi_pend_D.*THE_Theta_pend_D.*cos(THE_Psi_pend).*sin(THE_Theta_pend)-THE_Phi_D.*THE_Theta_D.*cos(THE_Theta).*(sin(THE_Phi_pend).*sin(THE_Psi_pend)+cos(THE_Phi_pend).*cos(THE_Psi_pend).*sin(THE_Theta_pend)))+m_pend.*(Lx_pend.^2./1.2e+1+Ly_pend.^2./1.2e+1).*(cos(THE_Psi).*(cos(THE_Phi_pend).*sin(THE_Psi_pend)-cos(THE_Psi_pend).*sin(THE_Phi_pend).*sin(THE_Theta_pend))+cos(THE_Psi_pend).*cos(THE_Theta_pend).*sin(THE_Psi)).*(((THE_Theta_D.*cos(THE_Psi)+THE_Phi_D.*cos(THE_Theta).*sin(THE_Psi)).*(-THE_Psi_pend_D.*cos(THE_Phi_pend).*cos(THE_Psi_pend)+THE_Phi_pend_D.*sin(THE_Phi_pend).*sin(THE_Psi_pend)-THE_Psi_pend_D.*sin(THE_Phi_pend).*sin(THE_Psi_pend).*sin(THE_Theta_pend)+THE_Phi_pend_D.*cos(THE_Phi_pend).*cos(THE_Psi_pend).*sin(THE_Theta_pend)+THE_Theta_pend_D.*cos(THE_Psi_pend).*cos(THE_Theta_pend).*sin(THE_Phi_pend)))./2.0+((THE_Psi_D-THE_Phi_D.*sin(THE_Theta)).*(THE_Phi_pend_D.*cos(THE_Phi_pend).*sin(THE_Psi_pend)+THE_Psi_pend_D.*cos(THE_Psi_pend).*sin(THE_Phi_pend)+THE_Theta_pend_D.*cos(THE_Phi_pend).*cos(THE_Psi_pend).*cos(THE_Theta_pend)-THE_Phi_pend_D.*cos(THE_Psi_pend).*sin(THE_Phi_pend).*sin(THE_Theta_pend)-THE_Psi_pend_D.*cos(THE_Phi_pend).*sin(THE_Psi_pend).*sin(THE_Theta_pend)))./2.0+((cos(THE_Phi_pend).*sin(THE_Psi_pend)-cos(THE_Psi_pend).*sin(THE_Phi_pend).*sin(THE_Theta_pend)).*(THE_Psi_D.*THE_Theta_D.*sin(THE_Psi)-THE_Phi_D.*THE_Psi_D.*cos(THE_Psi).*cos(THE_Theta)+THE_Phi_D.*THE_Theta_D.*sin(THE_Psi).*sin(THE_Theta)))./2.0-(THE_Psi_pend_D.*THE_Theta_pend_D.*cos(THE_Psi_pend))./2.0-(cos(THE_Psi_pend).*cos(THE_Theta_pend).*(THE_Psi_D.*THE_Theta_D.*cos(THE_Psi)+THE_Phi_D.*THE_Psi_D.*cos(THE_Theta).*sin(THE_Psi)+THE_Phi_D.*THE_Theta_D.*cos(THE_Psi).*sin(THE_Theta)))./2.0+(THE_Psi_pend_D.*cos(THE_Theta_pend).*sin(THE_Psi_pend).*(THE_Theta_D.*sin(THE_Psi)-THE_Phi_D.*cos(THE_Psi).*cos(THE_Theta)))./2.0+(THE_Theta_pend_D.*cos(THE_Psi_pend).*sin(THE_Theta_pend).*(THE_Theta_D.*sin(THE_Psi)-THE_Phi_D.*cos(THE_Psi).*cos(THE_Theta)))./2.0-(THE_Phi_pend_D.*THE_Psi_pend_D.*cos(THE_Theta_pend).*sin(THE_Psi_pend))./2.0-(THE_Phi_pend_D.*THE_Theta_pend_D.*cos(THE_Psi_pend).*sin(THE_Theta_pend))./2.0-(THE_Phi_D.*THE_Theta_D.*cos(THE_Theta).*(sin(THE_Phi_pend).*sin(THE_Psi_pend)+cos(THE_Phi_pend).*cos(THE_Psi_pend).*sin(THE_Theta_pend)))./2.0)-THE_Phi_D.*cos(THE_Psi).*sin(THE_Theta).*(I_xz.*(THE_Psi_D./2.0-(THE_Phi_D.*sin(THE_Theta))./2.0)+I_yz.*((THE_Theta_D.*cos(THE_Psi))./2.0+(THE_Phi_D.*cos(THE_Theta).*sin(THE_Psi))./2.0)-I_zz.*((THE_Theta_D.*sin(THE_Psi))./2.0-(THE_Phi_D.*cos(THE_Psi).*cos(THE_Theta))./2.0))-THE_Phi_D.*sin(THE_Psi).*sin(THE_Theta).*(I_xy.*(THE_Psi_D./2.0-(THE_Phi_D.*sin(THE_Theta))./2.0)+I_yy.*((THE_Theta_D.*cos(THE_Psi))./2.0+(THE_Phi_D.*cos(THE_Theta).*sin(THE_Psi))./2.0)-I_yz.*((THE_Theta_D.*sin(THE_Psi))./2.0-(THE_Phi_D.*cos(THE_Psi).*cos(THE_Theta))./2.0))+(mprop.*sin(THE_Theta).*(THE_Psi_D.*cg_to_mot_L.*cos(THE_Psi)-THE_Psi_D.*cg_to_mot_H.*sin(THE_Psi)).*(THE_Z_D-sin(THE_Theta).*(cg_to_mot_H.*(THE_Theta_D.*cos(THE_Psi)+THE_Phi_D.*cos(THE_Theta).*sin(THE_Psi))+cg_to_mot_L.*(THE_Theta_D.*sin(THE_Psi)-THE_Phi_D.*cos(THE_Psi).*cos(THE_Theta)))+cg_to_mot_L.*cos(THE_Psi).*cos(THE_Theta).*(THE_Psi_D-THE_Phi_D.*sin(THE_Theta))-cg_to_mot_H.*cos(THE_Theta).*sin(THE_Psi).*(THE_Psi_D-THE_Phi_D.*sin(THE_Theta))))./2.0+m_pend.*(Lx_pend.^2./1.2e+1+Ly_pend.^2./1.2e+1).*((THE_Phi_D.*cos(THE_Theta).*(sin(THE_Phi_pend).*sin(THE_Psi_pend)+cos(THE_Phi_pend).*cos(THE_Psi_pend).*sin(THE_Theta_pend)))./2.0-(THE_Phi_D.*sin(THE_Psi).*sin(THE_Theta).*(cos(THE_Phi_pend).*sin(THE_Psi_pend)-cos(THE_Psi_pend).*sin(THE_Phi_pend).*sin(THE_Theta_pend)))./2.0+(THE_Phi_D.*cos(THE_Psi).*cos(THE_Psi_pend).*cos(THE_Theta_pend).*sin(THE_Theta))./2.0).*((cos(THE_Phi_pend).*sin(THE_Psi_pend)-cos(THE_Psi_pend).*sin(THE_Phi_pend).*sin(THE_Theta_pend)).*(THE_Theta_D.*cos(THE_Psi)+THE_Phi_D.*cos(THE_Theta).*sin(THE_Psi))-(THE_Psi_D-THE_Phi_D.*sin(THE_Theta)).*(sin(THE_Phi_pend).*sin(THE_Psi_pend)+cos(THE_Phi_pend).*cos(THE_Psi_pend).*sin(THE_Theta_pend))+THE_Theta_pend_D.*sin(THE_Psi_pend)-THE_Phi_pend_D.*cos(THE_Psi_pend).*cos(THE_Theta_pend)+cos(THE_Psi_pend).*cos(THE_Theta_pend).*(THE_Theta_D.*sin(THE_Psi)-THE_Phi_D.*cos(THE_Psi).*cos(THE_Theta)))+m_pend.*(Lx_pend.^2./1.2e+1+Ly_pend.^2./1.2e+1).*(THE_Phi_D.*cos(THE_Theta).*(sin(THE_Phi_pend).*sin(THE_Psi_pend)+cos(THE_Phi_pend).*cos(THE_Psi_pend).*sin(THE_Theta_pend))-THE_Phi_D.*sin(THE_Psi).*sin(THE_Theta).*(cos(THE_Phi_pend).*sin(THE_Psi_pend)-cos(THE_Psi_pend).*sin(THE_Phi_pend).*sin(THE_Theta_pend))+THE_Phi_D.*cos(THE_Psi).*cos(THE_Psi_pend).*cos(THE_Theta_pend).*sin(THE_Theta)).*(((cos(THE_Phi_pend).*sin(THE_Psi_pend)-cos(THE_Psi_pend).*sin(THE_Phi_pend).*sin(THE_Theta_pend)).*(THE_Theta_D.*cos(THE_Psi)+THE_Phi_D.*cos(THE_Theta).*sin(THE_Psi)))./2.0-((THE_Psi_D-THE_Phi_D.*sin(THE_Theta)).*(sin(THE_Phi_pend).*sin(THE_Psi_pend)+cos(THE_Phi_pend).*cos(THE_Psi_pend).*sin(THE_Theta_pend)))./2.0+(THE_Theta_pend_D.*sin(THE_Psi_pend))./2.0-(THE_Phi_pend_D.*cos(THE_Psi_pend).*cos(THE_Theta_pend))./2.0+(cos(THE_Psi_pend).*cos(THE_Theta_pend).*(THE_Theta_D.*sin(THE_Psi)-THE_Phi_D.*cos(THE_Psi).*cos(THE_Theta)))./2.0)+m_pend.*(Lx_pend.^2./1.2e+1+Lz_pend.^2./1.2e+1).*(-cos(THE_Psi).*(-THE_Phi_pend_D.*cos(THE_Psi_pend).*sin(THE_Phi_pend)-THE_Psi_pend_D.*cos(THE_Phi_pend).*sin(THE_Psi_pend)+THE_Phi_pend_D.*cos(THE_Phi_pend).*sin(THE_Psi_pend).*sin(THE_Theta_pend)+THE_Psi_pend_D.*cos(THE_Psi_pend).*sin(THE_Phi_pend).*sin(THE_Theta_pend)+THE_Theta_pend_D.*cos(THE_Theta_pend).*sin(THE_Phi_pend).*sin(THE_Psi_pend))+THE_Psi_D.*sin(THE_Psi).*(cos(THE_Phi_pend).*cos(THE_Psi_pend)+sin(THE_Phi_pend).*sin(THE_Psi_pend).*sin(THE_Theta_pend))-THE_Theta_pend_D.*sin(THE_Psi).*sin(THE_Psi_pend).*sin(THE_Theta_pend)+THE_Psi_D.*cos(THE_Psi).*cos(THE_Theta_pend).*sin(THE_Psi_pend)+THE_Psi_pend_D.*cos(THE_Psi_pend).*cos(THE_Theta_pend).*sin(THE_Psi)).*(((cos(THE_Phi_pend).*cos(THE_Psi_pend)+sin(THE_Phi_pend).*sin(THE_Psi_pend).*sin(THE_Theta_pend)).*(THE_Theta_D.*cos(THE_Psi)+THE_Phi_D.*cos(THE_Theta).*sin(THE_Psi)))./2.0+(THE_Theta_pend_D.*cos(THE_Psi_pend))./2.0-((THE_Psi_D-THE_Phi_D.*sin(THE_Theta)).*(cos(THE_Psi_pend).*sin(THE_Phi_pend)-cos(THE_Phi_pend).*sin(THE_Psi_pend).*sin(THE_Theta_pend)))./2.0+(THE_Phi_pend_D.*cos(THE_Theta_pend).*sin(THE_Psi_pend))./2.0-(cos(THE_Theta_pend).*sin(THE_Psi_pend).*(THE_Theta_D.*sin(THE_Psi)-THE_Phi_D.*cos(THE_Psi).*cos(THE_Theta)))./2.0)+m_pend.*(Lx_pend.^2./1.2e+1+Lz_pend.^2./1.2e+1).*(cos(THE_Psi).*(-THE_Phi_pend_D.*cos(THE_Psi_pend).*sin(THE_Phi_pend)-THE_Psi_pend_D.*cos(THE_Phi_pend).*sin(THE_Psi_pend)+THE_Phi_pend_D.*cos(THE_Phi_pend).*sin(THE_Psi_pend).*sin(THE_Theta_pend)+THE_Psi_pend_D.*cos(THE_Psi_pend).*sin(THE_Phi_pend).*sin(THE_Theta_pend)+THE_Theta_pend_D.*cos(THE_Theta_pend).*sin(THE_Phi_pend).*sin(THE_Psi_pend)).*(-1.0./2.0)+(THE_Psi_D.*sin(THE_Psi).*(cos(THE_Phi_pend).*cos(THE_Psi_pend)+sin(THE_Phi_pend).*sin(THE_Psi_pend).*sin(THE_Theta_pend)))./2.0-(THE_Theta_pend_D.*sin(THE_Psi).*sin(THE_Psi_pend).*sin(THE_Theta_pend))./2.0+(THE_Psi_D.*cos(THE_Psi).*cos(THE_Theta_pend).*sin(THE_Psi_pend))./2.0+(THE_Psi_pend_D.*cos(THE_Psi_pend).*cos(THE_Theta_pend).*sin(THE_Psi))./2.0).*((cos(THE_Phi_pend).*cos(THE_Psi_pend)+sin(THE_Phi_pend).*sin(THE_Psi_pend).*sin(THE_Theta_pend)).*(THE_Theta_D.*cos(THE_Psi)+THE_Phi_D.*cos(THE_Theta).*sin(THE_Psi))+THE_Theta_pend_D.*cos(THE_Psi_pend)-(THE_Psi_D-THE_Phi_D.*sin(THE_Theta)).*(cos(THE_Psi_pend).*sin(THE_Phi_pend)-cos(THE_Phi_pend).*sin(THE_Psi_pend).*sin(THE_Theta_pend))+THE_Phi_pend_D.*cos(THE_Theta_pend).*sin(THE_Psi_pend)-cos(THE_Theta_pend).*sin(THE_Psi_pend).*(THE_Theta_D.*sin(THE_Psi)-THE_Phi_D.*cos(THE_Psi).*cos(THE_Theta)))-m_pend.*(Lx_pend.^2./1.2e+1+Lz_pend.^2./1.2e+1).*(THE_Phi_D.*cos(THE_Theta).*(cos(THE_Psi_pend).*sin(THE_Phi_pend)-cos(THE_Phi_pend).*sin(THE_Psi_pend).*sin(THE_Theta_pend)).*(-1.0./2.0)+(THE_Phi_D.*sin(THE_Psi).*sin(THE_Theta).*(cos(THE_Phi_pend).*cos(THE_Psi_pend)+sin(THE_Phi_pend).*sin(THE_Psi_pend).*sin(THE_Theta_pend)))./2.0+(THE_Phi_D.*cos(THE_Psi).*cos(THE_Theta_pend).*sin(THE_Theta).*sin(THE_Psi_pend))./2.0).*((cos(THE_Phi_pend).*cos(THE_Psi_pend)+sin(THE_Phi_pend).*sin(THE_Psi_pend).*sin(THE_Theta_pend)).*(THE_Theta_D.*cos(THE_Psi)+THE_Phi_D.*cos(THE_Theta).*sin(THE_Psi))+THE_Theta_pend_D.*cos(THE_Psi_pend)-(THE_Psi_D-THE_Phi_D.*sin(THE_Theta)).*(cos(THE_Psi_pend).*sin(THE_Phi_pend)-cos(THE_Phi_pend).*sin(THE_Psi_pend).*sin(THE_Theta_pend))+THE_Phi_pend_D.*cos(THE_Theta_pend).*sin(THE_Psi_pend)-cos(THE_Theta_pend).*sin(THE_Psi_pend).*(THE_Theta_D.*sin(THE_Psi)-THE_Phi_D.*cos(THE_Psi).*cos(THE_Theta)))-m_pend.*(Lx_pend.^2./1.2e+1+Lz_pend.^2./1.2e+1).*(-THE_Phi_D.*cos(THE_Theta).*(cos(THE_Psi_pend).*sin(THE_Phi_pend)-cos(THE_Phi_pend).*sin(THE_Psi_pend).*sin(THE_Theta_pend))+THE_Phi_D.*sin(THE_Psi).*sin(THE_Theta).*(cos(THE_Phi_pend).*cos(THE_Psi_pend)+sin(THE_Phi_pend).*sin(THE_Psi_pend).*sin(THE_Theta_pend))+THE_Phi_D.*cos(THE_Psi).*cos(THE_Theta_pend).*sin(THE_Theta).*sin(THE_Psi_pend)).*(((cos(THE_Phi_pend).*cos(THE_Psi_pend)+sin(THE_Phi_pend).*sin(THE_Psi_pend).*sin(THE_Theta_pend)).*(THE_Theta_D.*cos(THE_Psi)+THE_Phi_D.*cos(THE_Theta).*sin(THE_Psi)))./2.0+(THE_Theta_pend_D.*cos(THE_Psi_pend))./2.0-((THE_Psi_D-THE_Phi_D.*sin(THE_Theta)).*(cos(THE_Psi_pend).*sin(THE_Phi_pend)-cos(THE_Phi_pend).*sin(THE_Psi_pend).*sin(THE_Theta_pend)))./2.0+(THE_Phi_pend_D.*cos(THE_Theta_pend).*sin(THE_Psi_pend))./2.0-(cos(THE_Theta_pend).*sin(THE_Psi_pend).*(THE_Theta_D.*sin(THE_Psi)-THE_Phi_D.*cos(THE_Psi).*cos(THE_Theta)))./2.0)-m_pend.*((cos(THE_Psi).*(cos(THE_Phi_pend).*cos(THE_Psi_pend)+sin(THE_Phi_pend).*sin(THE_Psi_pend).*sin(THE_Theta_pend)))./2.0-(cos(THE_Theta_pend).*sin(THE_Psi).*sin(THE_Psi_pend))./2.0).*(Lx_pend.^2./1.2e+1+Lz_pend.^2./1.2e+1).*((THE_Theta_D.*cos(THE_Psi)+THE_Phi_D.*cos(THE_Theta).*sin(THE_Psi)).*(-THE_Phi_pend_D.*cos(THE_Psi_pend).*sin(THE_Phi_pend)-THE_Psi_pend_D.*cos(THE_Phi_pend).*sin(THE_Psi_pend)+THE_Phi_pend_D.*cos(THE_Phi_pend).*sin(THE_Psi_pend).*sin(THE_Theta_pend)+THE_Psi_pend_D.*cos(THE_Psi_pend).*sin(THE_Phi_pend).*sin(THE_Theta_pend)+THE_Theta_pend_D.*cos(THE_Theta_pend).*sin(THE_Phi_pend).*sin(THE_Psi_pend))+(THE_Psi_D-THE_Phi_D.*sin(THE_Theta)).*(-THE_Phi_pend_D.*cos(THE_Phi_pend).*cos(THE_Psi_pend)+THE_Psi_pend_D.*sin(THE_Phi_pend).*sin(THE_Psi_pend)-THE_Phi_pend_D.*sin(THE_Phi_pend).*sin(THE_Psi_pend).*sin(THE_Theta_pend)+THE_Psi_pend_D.*cos(THE_Phi_pend).*cos(THE_Psi_pend).*sin(THE_Theta_pend)+THE_Theta_pend_D.*cos(THE_Phi_pend).*cos(THE_Theta_pend).*sin(THE_Psi_pend))-(cos(THE_Phi_pend).*cos(THE_Psi_pend)+sin(THE_Phi_pend).*sin(THE_Psi_pend).*sin(THE_Theta_pend)).*(THE_Psi_D.*THE_Theta_D.*sin(THE_Psi)-THE_Phi_D.*THE_Psi_D.*cos(THE_Psi).*cos(THE_Theta)+THE_Phi_D.*THE_Theta_D.*sin(THE_Psi).*sin(THE_Theta))-cos(THE_Theta_pend).*sin(THE_Psi_pend).*(THE_Psi_D.*THE_Theta_D.*cos(THE_Psi)+THE_Phi_D.*THE_Psi_D.*cos(THE_Theta).*sin(THE_Psi)+THE_Phi_D.*THE_Theta_D.*cos(THE_Psi).*sin(THE_Theta))-THE_Psi_pend_D.*THE_Theta_pend_D.*sin(THE_Psi_pend)-THE_Psi_pend_D.*cos(THE_Psi_pend).*cos(THE_Theta_pend).*(THE_Theta_D.*sin(THE_Psi)-THE_Phi_D.*cos(THE_Psi).*cos(THE_Theta))+THE_Theta_pend_D.*sin(THE_Psi_pend).*sin(THE_Theta_pend).*(THE_Theta_D.*sin(THE_Psi)-THE_Phi_D.*cos(THE_Psi).*cos(THE_Theta))+THE_Phi_pend_D.*THE_Psi_pend_D.*cos(THE_Psi_pend).*cos(THE_Theta_pend)-THE_Phi_pend_D.*THE_Theta_pend_D.*sin(THE_Psi_pend).*sin(THE_Theta_pend)+THE_Phi_D.*THE_Theta_D.*cos(THE_Theta).*(cos(THE_Psi_pend).*sin(THE_Phi_pend)-cos(THE_Phi_pend).*sin(THE_Psi_pend).*sin(THE_Theta_pend)))-m_pend.*(cos(THE_Psi).*(cos(THE_Phi_pend).*cos(THE_Psi_pend)+sin(THE_Phi_pend).*sin(THE_Psi_pend).*sin(THE_Theta_pend))-cos(THE_Theta_pend).*sin(THE_Psi).*sin(THE_Psi_pend)).*(Lx_pend.^2./1.2e+1+Lz_pend.^2./1.2e+1).*(((THE_Theta_D.*cos(THE_Psi)+THE_Phi_D.*cos(THE_Theta).*sin(THE_Psi)).*(-THE_Phi_pend_D.*cos(THE_Psi_pend).*sin(THE_Phi_pend)-THE_Psi_pend_D.*cos(THE_Phi_pend).*sin(THE_Psi_pend)+THE_Phi_pend_D.*cos(THE_Phi_pend).*sin(THE_Psi_pend).*sin(THE_Theta_pend)+THE_Psi_pend_D.*cos(THE_Psi_pend).*sin(THE_Phi_pend).*sin(THE_Theta_pend)+THE_Theta_pend_D.*cos(THE_Theta_pend).*sin(THE_Phi_pend).*sin(THE_Psi_pend)))./2.0+((THE_Psi_D-THE_Phi_D.*sin(THE_Theta)).*(-THE_Phi_pend_D.*cos(THE_Phi_pend).*cos(THE_Psi_pend)+THE_Psi_pend_D.*sin(THE_Phi_pend).*sin(THE_Psi_pend)-THE_Phi_pend_D.*sin(THE_Phi_pend).*sin(THE_Psi_pend).*sin(THE_Theta_pend)+THE_Psi_pend_D.*cos(THE_Phi_pend).*cos(THE_Psi_pend).*sin(THE_Theta_pend)+THE_Theta_pend_D.*cos(THE_Phi_pend).*cos(THE_Theta_pend).*sin(THE_Psi_pend)))./2.0-((cos(THE_Phi_pend).*cos(THE_Psi_pend)+sin(THE_Phi_pend).*sin(THE_Psi_pend).*sin(THE_Theta_pend)).*(THE_Psi_D.*THE_Theta_D.*sin(THE_Psi)-THE_Phi_D.*THE_Psi_D.*cos(THE_Psi).*cos(THE_Theta)+THE_Phi_D.*THE_Theta_D.*sin(THE_Psi).*sin(THE_Theta)))./2.0-(cos(THE_Theta_pend).*sin(THE_Psi_pend).*(THE_Psi_D.*THE_Theta_D.*cos(THE_Psi)+THE_Phi_D.*THE_Psi_D.*cos(THE_Theta).*sin(THE_Psi)+THE_Phi_D.*THE_Theta_D.*cos(THE_Psi).*sin(THE_Theta)))./2.0-(THE_Psi_pend_D.*THE_Theta_pend_D.*sin(THE_Psi_pend))./2.0-(THE_Psi_pend_D.*cos(THE_Psi_pend).*cos(THE_Theta_pend).*(THE_Theta_D.*sin(THE_Psi)-THE_Phi_D.*cos(THE_Psi).*cos(THE_Theta)))./2.0+(THE_Theta_pend_D.*sin(THE_Psi_pend).*sin(THE_Theta_pend).*(THE_Theta_D.*sin(THE_Psi)-THE_Phi_D.*cos(THE_Psi).*cos(THE_Theta)))./2.0+(THE_Phi_pend_D.*THE_Psi_pend_D.*cos(THE_Psi_pend).*cos(THE_Theta_pend))./2.0-(THE_Phi_pend_D.*THE_Theta_pend_D.*sin(THE_Psi_pend).*sin(THE_Theta_pend))./2.0+(THE_Phi_D.*THE_Theta_D.*cos(THE_Theta).*(cos(THE_Psi_pend).*sin(THE_Phi_pend)-cos(THE_Phi_pend).*sin(THE_Psi_pend).*sin(THE_Theta_pend)))./2.0)-m_pend.*(Ly_pend.^2./1.2e+1+Lz_pend.^2./1.2e+1).*(THE_Psi_pend_D./2.0+(sin(THE_Theta_pend).*(THE_Theta_D.*sin(THE_Psi)-THE_Phi_D.*cos(THE_Psi).*cos(THE_Theta)))./2.0-(THE_Phi_pend_D.*sin(THE_Theta_pend))./2.0+(cos(THE_Theta_pend).*sin(THE_Phi_pend).*(THE_Theta_D.*cos(THE_Psi)+THE_Phi_D.*cos(THE_Theta).*sin(THE_Psi)))./2.0+(cos(THE_Phi_pend).*cos(THE_Theta_pend).*(THE_Psi_D-THE_Phi_D.*sin(THE_Theta)))./2.0).*(THE_Psi_D.*cos(THE_Psi).*sin(THE_Theta_pend)+THE_Theta_pend_D.*cos(THE_Theta_pend).*sin(THE_Psi)+THE_Phi_pend_D.*cos(THE_Psi).*cos(THE_Phi_pend).*cos(THE_Theta_pend)-THE_Psi_D.*cos(THE_Theta_pend).*sin(THE_Psi).*sin(THE_Phi_pend)-THE_Theta_pend_D.*cos(THE_Psi).*sin(THE_Phi_pend).*sin(THE_Theta_pend))-m_pend.*(Ly_pend.^2./1.2e+1+Lz_pend.^2./1.2e+1).*((THE_Phi_D.*cos(THE_Theta).*cos(THE_Phi_pend).*cos(THE_Theta_pend))./2.0-(THE_Phi_D.*cos(THE_Psi).*sin(THE_Theta).*sin(THE_Theta_pend))./2.0+(THE_Phi_D.*cos(THE_Theta_pend).*sin(THE_Psi).*sin(THE_Theta).*sin(THE_Phi_pend))./2.0).*(THE_Psi_pend_D+sin(THE_Theta_pend).*(THE_Theta_D.*sin(THE_Psi)-THE_Phi_D.*cos(THE_Psi).*cos(THE_Theta))-THE_Phi_pend_D.*sin(THE_Theta_pend)+cos(THE_Theta_pend).*sin(THE_Phi_pend).*(THE_Theta_D.*cos(THE_Psi)+THE_Phi_D.*cos(THE_Theta).*sin(THE_Psi))+cos(THE_Phi_pend).*cos(THE_Theta_pend).*(THE_Psi_D-THE_Phi_D.*sin(THE_Theta)))+m_pend.*(Ly_pend.^2./1.2e+1+Lz_pend.^2./1.2e+1).*((sin(THE_Psi).*sin(THE_Theta_pend))./2.0+(cos(THE_Psi).*cos(THE_Theta_pend).*sin(THE_Phi_pend))./2.0).*(-sin(THE_Theta_pend).*(THE_Psi_D.*THE_Theta_D.*cos(THE_Psi)+THE_Phi_D.*THE_Psi_D.*cos(THE_Theta).*sin(THE_Psi)+THE_Phi_D.*THE_Theta_D.*cos(THE_Psi).*sin(THE_Theta))+cos(THE_Theta_pend).*sin(THE_Phi_pend).*(THE_Psi_D.*THE_Theta_D.*sin(THE_Psi)-THE_Phi_D.*THE_Psi_D.*cos(THE_Psi).*cos(THE_Theta)+THE_Phi_D.*THE_Theta_D.*sin(THE_Psi).*sin(THE_Theta))-THE_Theta_pend_D.*cos(THE_Theta_pend).*(THE_Theta_D.*sin(THE_Psi)-THE_Phi_D.*cos(THE_Psi).*cos(THE_Theta))+THE_Phi_pend_D.*THE_Theta_pend_D.*cos(THE_Theta_pend)-THE_Phi_pend_D.*cos(THE_Phi_pend).*cos(THE_Theta_pend).*(THE_Theta_D.*cos(THE_Psi)+THE_Phi_D.*cos(THE_Theta).*sin(THE_Psi))+THE_Theta_pend_D.*sin(THE_Phi_pend).*sin(THE_Theta_pend).*(THE_Theta_D.*cos(THE_Psi)+THE_Phi_D.*cos(THE_Theta).*sin(THE_Psi))+THE_Phi_pend_D.*cos(THE_Theta_pend).*sin(THE_Phi_pend).*(THE_Psi_D-THE_Phi_D.*sin(THE_Theta))+THE_Theta_pend_D.*cos(THE_Phi_pend).*sin(THE_Theta_pend).*(THE_Psi_D-THE_Phi_D.*sin(THE_Theta))+THE_Phi_D.*THE_Theta_D.*cos(THE_Theta).*cos(THE_Phi_pend).*cos(THE_Theta_pend))+m_pend.*(Ly_pend.^2./1.2e+1+Lz_pend.^2./1.2e+1).*(sin(THE_Psi).*sin(THE_Theta_pend)+cos(THE_Psi).*cos(THE_Theta_pend).*sin(THE_Phi_pend)).*(sin(THE_Theta_pend).*(THE_Psi_D.*THE_Theta_D.*cos(THE_Psi)+THE_Phi_D.*THE_Psi_D.*cos(THE_Theta).*sin(THE_Psi)+THE_Phi_D.*THE_Theta_D.*cos(THE_Psi).*sin(THE_Theta)).*(-1.0./2.0)+(cos(THE_Theta_pend).*sin(THE_Phi_pend).*(THE_Psi_D.*THE_Theta_D.*sin(THE_Psi)-THE_Phi_D.*THE_Psi_D.*cos(THE_Psi).*cos(THE_Theta)+THE_Phi_D.*THE_Theta_D.*sin(THE_Psi).*sin(THE_Theta)))./2.0-(THE_Theta_pend_D.*cos(THE_Theta_pend).*(THE_Theta_D.*sin(THE_Psi)-THE_Phi_D.*cos(THE_Psi).*cos(THE_Theta)))./2.0+(THE_Phi_pend_D.*THE_Theta_pend_D.*cos(THE_Theta_pend))./2.0-(THE_Phi_pend_D.*cos(THE_Phi_pend).*cos(THE_Theta_pend).*(THE_Theta_D.*cos(THE_Psi)+THE_Phi_D.*cos(THE_Theta).*sin(THE_Psi)))./2.0+(THE_Theta_pend_D.*sin(THE_Phi_pend).*sin(THE_Theta_pend).*(THE_Theta_D.*cos(THE_Psi)+THE_Phi_D.*cos(THE_Theta).*sin(THE_Psi)))./2.0+(THE_Phi_pend_D.*cos(THE_Theta_pend).*sin(THE_Phi_pend).*(THE_Psi_D-THE_Phi_D.*sin(THE_Theta)))./2.0+(THE_Theta_pend_D.*cos(THE_Phi_pend).*sin(THE_Theta_pend).*(THE_Psi_D-THE_Phi_D.*sin(THE_Theta)))./2.0+(THE_Phi_D.*THE_Theta_D.*cos(THE_Theta).*cos(THE_Phi_pend).*cos(THE_Theta_pend))./2.0)+(mprop.*sin(THE_Theta).*(THE_Psi_D.*cg_to_mot_L.*cos(THE_Psi)+THE_Psi_D.*cg_to_mot_H.*sin(THE_Psi)).*(-THE_Z_D+sin(THE_Theta).*(cg_to_mot_H.*(THE_Theta_D.*cos(THE_Psi)+THE_Phi_D.*cos(THE_Theta).*sin(THE_Psi))-cg_to_mot_L.*(THE_Theta_D.*sin(THE_Psi)-THE_Phi_D.*cos(THE_Psi).*cos(THE_Theta)))+cg_to_mot_L.*cos(THE_Psi).*cos(THE_Theta).*(THE_Psi_D-THE_Phi_D.*sin(THE_Theta))+cg_to_mot_H.*cos(THE_Theta).*sin(THE_Psi).*(THE_Psi_D-THE_Phi_D.*sin(THE_Theta))))./2.0+mprop.*sin(THE_Theta).*(THE_Psi_D.*cg_to_mot_L.*cos(THE_Psi)+THE_Psi_D.*cg_to_mot_H.*sin(THE_Psi)).*(THE_Z_D.*(-1.0./2.0)+(sin(THE_Theta).*(cg_to_mot_H.*(THE_Theta_D.*cos(THE_Psi)+THE_Phi_D.*cos(THE_Theta).*sin(THE_Psi))-cg_to_mot_L.*(THE_Theta_D.*sin(THE_Psi)-THE_Phi_D.*cos(THE_Psi).*cos(THE_Theta))))./2.0+(cg_to_mot_L.*cos(THE_Psi).*cos(THE_Theta).*(THE_Psi_D-THE_Phi_D.*sin(THE_Theta)))./2.0+(cg_to_mot_H.*cos(THE_Theta).*sin(THE_Psi).*(THE_Psi_D-THE_Phi_D.*sin(THE_Theta)))./2.0)+mprop.*sin(THE_Theta).*(THE_Psi_D.*cg_to_mot_L.*cos(THE_Psi)-THE_Psi_D.*cg_to_mot_H.*sin(THE_Psi)).*(THE_Z_D./2.0-(sin(THE_Theta).*(cg_to_mot_H.*(THE_Theta_D.*cos(THE_Psi)+THE_Phi_D.*cos(THE_Theta).*sin(THE_Psi))+cg_to_mot_L.*(THE_Theta_D.*sin(THE_Psi)-THE_Phi_D.*cos(THE_Psi).*cos(THE_Theta))))./2.0+(cg_to_mot_L.*cos(THE_Psi).*cos(THE_Theta).*(THE_Psi_D-THE_Phi_D.*sin(THE_Theta)))./2.0-(cg_to_mot_H.*cos(THE_Theta).*sin(THE_Psi).*(THE_Psi_D-THE_Phi_D.*sin(THE_Theta)))./2.0)-(mprop.*sin(THE_Theta).*(cg_to_mot_H.*cos(THE_Psi)+cg_to_mot_L.*sin(THE_Psi)).*(-sin(THE_Theta).*(cg_to_mot_H.*(THE_Psi_D.*THE_Theta_D.*sin(THE_Psi)-THE_Phi_D.*THE_Psi_D.*cos(THE_Psi).*cos(THE_Theta)+THE_Phi_D.*THE_Theta_D.*sin(THE_Psi).*sin(THE_Theta))-cg_to_mot_L.*(THE_Psi_D.*THE_Theta_D.*cos(THE_Psi)+THE_Phi_D.*THE_Psi_D.*cos(THE_Theta).*sin(THE_Psi)+THE_Phi_D.*THE_Theta_D.*cos(THE_Psi).*sin(THE_Theta)))+THE_Theta_D.*cos(THE_Theta).*(cg_to_mot_H.*(THE_Theta_D.*cos(THE_Psi)+THE_Phi_D.*cos(THE_Theta).*sin(THE_Psi))+cg_to_mot_L.*(THE_Theta_D.*sin(THE_Psi)-THE_Phi_D.*cos(THE_Psi).*cos(THE_Theta)))+THE_Phi_D.*THE_Theta_D.*cg_to_mot_L.*cos(THE_Psi).*cos(THE_Theta).^2-THE_Phi_D.*THE_Theta_D.*cg_to_mot_H.*cos(THE_Theta).^2.*sin(THE_Psi)+THE_Psi_D.*cg_to_mot_H.*cos(THE_Psi).*cos(THE_Theta).*(THE_Psi_D-THE_Phi_D.*sin(THE_Theta))+THE_Psi_D.*cg_to_mot_L.*cos(THE_Theta).*sin(THE_Psi).*(THE_Psi_D-THE_Phi_D.*sin(THE_Theta))+THE_Theta_D.*cg_to_mot_L.*cos(THE_Psi).*sin(THE_Theta).*(THE_Psi_D-THE_Phi_D.*sin(THE_Theta))-THE_Theta_D.*cg_to_mot_H.*sin(THE_Psi).*sin(THE_Theta).*(THE_Psi_D-THE_Phi_D.*sin(THE_Theta))))./2.0+(mprop.*sin(THE_Theta).*(cg_to_mot_H.*cos(THE_Psi)-cg_to_mot_L.*sin(THE_Psi)).*(sin(THE_Theta).*(cg_to_mot_H.*(THE_Psi_D.*THE_Theta_D.*sin(THE_Psi)-THE_Phi_D.*THE_Psi_D.*cos(THE_Psi).*cos(THE_Theta)+THE_Phi_D.*THE_Theta_D.*sin(THE_Psi).*sin(THE_Theta))+cg_to_mot_L.*(THE_Psi_D.*THE_Theta_D.*cos(THE_Psi)+THE_Phi_D.*THE_Psi_D.*cos(THE_Theta).*sin(THE_Psi)+THE_Phi_D.*THE_Theta_D.*cos(THE_Psi).*sin(THE_Theta)))-THE_Theta_D.*cos(THE_Theta).*(cg_to_mot_H.*(THE_Theta_D.*cos(THE_Psi)+THE_Phi_D.*cos(THE_Theta).*sin(THE_Psi))-cg_to_mot_L.*(THE_Theta_D.*sin(THE_Psi)-THE_Phi_D.*cos(THE_Psi).*cos(THE_Theta)))+THE_Phi_D.*THE_Theta_D.*cg_to_mot_L.*cos(THE_Psi).*cos(THE_Theta).^2+THE_Phi_D.*THE_Theta_D.*cg_to_mot_H.*cos(THE_Theta).^2.*sin(THE_Psi)-THE_Psi_D.*cg_to_mot_H.*cos(THE_Psi).*cos(THE_Theta).*(THE_Psi_D-THE_Phi_D.*sin(THE_Theta))+THE_Psi_D.*cg_to_mot_L.*cos(THE_Theta).*sin(THE_Psi).*(THE_Psi_D-THE_Phi_D.*sin(THE_Theta))+THE_Theta_D.*cg_to_mot_L.*cos(THE_Psi).*sin(THE_Theta).*(THE_Psi_D-THE_Phi_D.*sin(THE_Theta))+THE_Theta_D.*cg_to_mot_H.*sin(THE_Psi).*sin(THE_Theta).*(THE_Psi_D-THE_Phi_D.*sin(THE_Theta))))./2.0-mprop.*sin(THE_Theta).*(cg_to_mot_H.*cos(THE_Psi)+cg_to_mot_L.*sin(THE_Psi)).*(sin(THE_Theta).*(cg_to_mot_H.*(THE_Psi_D.*THE_Theta_D.*sin(THE_Psi)-THE_Phi_D.*THE_Psi_D.*cos(THE_Psi).*cos(THE_Theta)+THE_Phi_D.*THE_Theta_D.*sin(THE_Psi).*sin(THE_Theta))-cg_to_mot_L.*(THE_Psi_D.*THE_Theta_D.*cos(THE_Psi)+THE_Phi_D.*THE_Psi_D.*cos(THE_Theta).*sin(THE_Psi)+THE_Phi_D.*THE_Theta_D.*cos(THE_Psi).*sin(THE_Theta))).*(-1.0./2.0)+(THE_Theta_D.*cos(THE_Theta).*(cg_to_mot_H.*(THE_Theta_D.*cos(THE_Psi)+THE_Phi_D.*cos(THE_Theta).*sin(THE_Psi))+cg_to_mot_L.*(THE_Theta_D.*sin(THE_Psi)-THE_Phi_D.*cos(THE_Psi).*cos(THE_Theta))))./2.0+(THE_Phi_D.*THE_Theta_D.*cg_to_mot_L.*cos(THE_Psi).*cos(THE_Theta).^2)./2.0-(THE_Phi_D.*THE_Theta_D.*cg_to_mot_H.*cos(THE_Theta).^2.*sin(THE_Psi))./2.0+(THE_Psi_D.*cg_to_mot_H.*cos(THE_Psi).*cos(THE_Theta).*(THE_Psi_D-THE_Phi_D.*sin(THE_Theta)))./2.0+(THE_Psi_D.*cg_to_mot_L.*cos(THE_Theta).*sin(THE_Psi).*(THE_Psi_D-THE_Phi_D.*sin(THE_Theta)))./2.0+(THE_Theta_D.*cg_to_mot_L.*cos(THE_Psi).*sin(THE_Theta).*(THE_Psi_D-THE_Phi_D.*sin(THE_Theta)))./2.0-(THE_Theta_D.*cg_to_mot_H.*sin(THE_Psi).*sin(THE_Theta).*(THE_Psi_D-THE_Phi_D.*sin(THE_Theta)))./2.0)+mprop.*sin(THE_Theta).*(cg_to_mot_H.*cos(THE_Psi)-cg_to_mot_L.*sin(THE_Psi)).*((sin(THE_Theta).*(cg_to_mot_H.*(THE_Psi_D.*THE_Theta_D.*sin(THE_Psi)-THE_Phi_D.*THE_Psi_D.*cos(THE_Psi).*cos(THE_Theta)+THE_Phi_D.*THE_Theta_D.*sin(THE_Psi).*sin(THE_Theta))+cg_to_mot_L.*(THE_Psi_D.*THE_Theta_D.*cos(THE_Psi)+THE_Phi_D.*THE_Psi_D.*cos(THE_Theta).*sin(THE_Psi)+THE_Phi_D.*THE_Theta_D.*cos(THE_Psi).*sin(THE_Theta))))./2.0-(THE_Theta_D.*cos(THE_Theta).*(cg_to_mot_H.*(THE_Theta_D.*cos(THE_Psi)+THE_Phi_D.*cos(THE_Theta).*sin(THE_Psi))-cg_to_mot_L.*(THE_Theta_D.*sin(THE_Psi)-THE_Phi_D.*cos(THE_Psi).*cos(THE_Theta))))./2.0+(THE_Phi_D.*THE_Theta_D.*cg_to_mot_L.*cos(THE_Psi).*cos(THE_Theta).^2)./2.0+(THE_Phi_D.*THE_Theta_D.*cg_to_mot_H.*cos(THE_Theta).^2.*sin(THE_Psi))./2.0-(THE_Psi_D.*cg_to_mot_H.*cos(THE_Psi).*cos(THE_Theta).*(THE_Psi_D-THE_Phi_D.*sin(THE_Theta)))./2.0+(THE_Psi_D.*cg_to_mot_L.*cos(THE_Theta).*sin(THE_Psi).*(THE_Psi_D-THE_Phi_D.*sin(THE_Theta)))./2.0+(THE_Theta_D.*cg_to_mot_L.*cos(THE_Psi).*sin(THE_Theta).*(THE_Psi_D-THE_Phi_D.*sin(THE_Theta)))./2.0+(THE_Theta_D.*cg_to_mot_H.*sin(THE_Psi).*sin(THE_Theta).*(THE_Psi_D-THE_Phi_D.*sin(THE_Theta)))./2.0)-m_pend.*(Ly_pend.^2./1.2e+1+Lz_pend.^2./1.2e+1).*(THE_Phi_D.*cos(THE_Theta).*cos(THE_Phi_pend).*cos(THE_Theta_pend)-THE_Phi_D.*cos(THE_Psi).*sin(THE_Theta).*sin(THE_Theta_pend)+THE_Phi_D.*cos(THE_Theta_pend).*sin(THE_Psi).*sin(THE_Theta).*sin(THE_Phi_pend)).*(THE_Psi_pend_D./2.0+(sin(THE_Theta_pend).*(THE_Theta_D.*sin(THE_Psi)-THE_Phi_D.*cos(THE_Psi).*cos(THE_Theta)))./2.0-(THE_Phi_pend_D.*sin(THE_Theta_pend))./2.0+(cos(THE_Theta_pend).*sin(THE_Phi_pend).*(THE_Theta_D.*cos(THE_Psi)+THE_Phi_D.*cos(THE_Theta).*sin(THE_Psi)))./2.0+(cos(THE_Phi_pend).*cos(THE_Theta_pend).*(THE_Psi_D-THE_Phi_D.*sin(THE_Theta)))./2.0)-THE_Phi_D.*cos(THE_Psi).*sin(THE_Theta).*(Iprop_xz.*(THE_Psi_D./2.0-(THE_Phi_D.*sin(THE_Theta))./2.0)+Iprop_zz.*(wMOT_1./2.0-(THE_Theta_D.*sin(THE_Psi))./2.0+(THE_Phi_D.*cos(THE_Psi).*cos(THE_Theta))./2.0)+Iprop_yz.*((THE_Theta_D.*cos(THE_Psi))./2.0+(THE_Phi_D.*cos(THE_Theta).*sin(THE_Psi))./2.0))-THE_Phi_D.*cos(THE_Psi).*sin(THE_Theta).*(Iprop_xz.*(THE_Psi_D./2.0-(THE_Phi_D.*sin(THE_Theta))./2.0)+Iprop_zz.*(wMOT_2./2.0-(THE_Theta_D.*sin(THE_Psi))./2.0+(THE_Phi_D.*cos(THE_Psi).*cos(THE_Theta))./2.0)+Iprop_yz.*((THE_Theta_D.*cos(THE_Psi))./2.0+(THE_Phi_D.*cos(THE_Theta).*sin(THE_Psi))./2.0))-THE_Phi_D.*cos(THE_Psi).*sin(THE_Theta).*(Iprop_xz.*(THE_Psi_D./2.0-(THE_Phi_D.*sin(THE_Theta))./2.0)+Iprop_zz.*(wMOT_3./2.0-(THE_Theta_D.*sin(THE_Psi))./2.0+(THE_Phi_D.*cos(THE_Psi).*cos(THE_Theta))./2.0)+Iprop_yz.*((THE_Theta_D.*cos(THE_Psi))./2.0+(THE_Phi_D.*cos(THE_Theta).*sin(THE_Psi))./2.0))-THE_Phi_D.*cos(THE_Psi).*sin(THE_Theta).*(Iprop_xz.*(THE_Psi_D./2.0-(THE_Phi_D.*sin(THE_Theta))./2.0)+Iprop_zz.*(wMOT_4./2.0-(THE_Theta_D.*sin(THE_Psi))./2.0+(THE_Phi_D.*cos(THE_Psi).*cos(THE_Theta))./2.0)+Iprop_yz.*((THE_Theta_D.*cos(THE_Psi))./2.0+(THE_Phi_D.*cos(THE_Theta).*sin(THE_Psi))./2.0))+THE_Phi_D.*THE_Theta_D.*cos(THE_Theta).*((I_xy.*cos(THE_Psi))./2.0-(I_xz.*sin(THE_Psi))./2.0)+THE_Phi_D.*THE_Theta_D.*cos(THE_Theta).*((Iprop_xy.*cos(THE_Psi))./2.0-(Iprop_xz.*sin(THE_Psi))./2.0).*4.0-Tbz_1.*cos(THE_Psi).*cos(THE_Theta).*(cg_to_mot_H.*cos(THE_Psi).*sin(THE_Theta)+cg_to_mot_L.*cos(THE_Psi).^2.*cos(THE_Theta)+cg_to_mot_L.*cos(THE_Theta).*sin(THE_Psi).^2)+Tbz_3.*cos(THE_Psi).*cos(THE_Theta).*(-cg_to_mot_H.*cos(THE_Psi).*sin(THE_Theta)+cg_to_mot_L.*cos(THE_Psi).^2.*cos(THE_Theta)+cg_to_mot_L.*cos(THE_Theta).*sin(THE_Psi).^2)-THE_Phi_D.*sin(THE_Psi).*sin(THE_Theta).*(Iprop_xy.*(THE_Psi_D./2.0-(THE_Phi_D.*sin(THE_Theta))./2.0)+Iprop_yz.*(wMOT_1./2.0-(THE_Theta_D.*sin(THE_Psi))./2.0+(THE_Phi_D.*cos(THE_Psi).*cos(THE_Theta))./2.0)+Iprop_yy.*((THE_Theta_D.*cos(THE_Psi))./2.0+(THE_Phi_D.*cos(THE_Theta).*sin(THE_Psi))./2.0))-THE_Phi_D.*sin(THE_Psi).*sin(THE_Theta).*(Iprop_xy.*(THE_Psi_D./2.0-(THE_Phi_D.*sin(THE_Theta))./2.0)+Iprop_yz.*(wMOT_2./2.0-(THE_Theta_D.*sin(THE_Psi))./2.0+(THE_Phi_D.*cos(THE_Psi).*cos(THE_Theta))./2.0)+Iprop_yy.*((THE_Theta_D.*cos(THE_Psi))./2.0+(THE_Phi_D.*cos(THE_Theta).*sin(THE_Psi))./2.0))-THE_Phi_D.*sin(THE_Psi).*sin(THE_Theta).*(Iprop_xy.*(THE_Psi_D./2.0-(THE_Phi_D.*sin(THE_Theta))./2.0)+Iprop_yz.*(wMOT_3./2.0-(THE_Theta_D.*sin(THE_Psi))./2.0+(THE_Phi_D.*cos(THE_Psi).*cos(THE_Theta))./2.0)+Iprop_yy.*((THE_Theta_D.*cos(THE_Psi))./2.0+(THE_Phi_D.*cos(THE_Theta).*sin(THE_Psi))./2.0))-THE_Phi_D.*sin(THE_Psi).*sin(THE_Theta).*(Iprop_xy.*(THE_Psi_D./2.0-(THE_Phi_D.*sin(THE_Theta))./2.0)+Iprop_yz.*(wMOT_4./2.0-(THE_Theta_D.*sin(THE_Psi))./2.0+(THE_Phi_D.*cos(THE_Psi).*cos(THE_Theta))./2.0)+Iprop_yy.*((THE_Theta_D.*cos(THE_Psi))./2.0+(THE_Phi_D.*cos(THE_Theta).*sin(THE_Psi))./2.0))-(THE_Theta_D.*mprop.*cos(THE_Theta).*(cg_to_mot_H.*cos(THE_Psi)-cg_to_mot_L.*sin(THE_Psi)).*(-THE_Z_D+sin(THE_Theta).*(cg_to_mot_H.*(THE_Theta_D.*cos(THE_Psi)+THE_Phi_D.*cos(THE_Theta).*sin(THE_Psi))-cg_to_mot_L.*(THE_Theta_D.*sin(THE_Psi)-THE_Phi_D.*cos(THE_Psi).*cos(THE_Theta)))+cg_to_mot_L.*cos(THE_Psi).*cos(THE_Theta).*(THE_Psi_D-THE_Phi_D.*sin(THE_Theta))+cg_to_mot_H.*cos(THE_Theta).*sin(THE_Psi).*(THE_Psi_D-THE_Phi_D.*sin(THE_Theta))))./2.0+THE_Theta_D.*mprop.*cos(THE_Theta).*(cg_to_mot_H.*cos(THE_Psi)+cg_to_mot_L.*sin(THE_Psi)).*(THE_Z_D./2.0-(sin(THE_Theta).*(cg_to_mot_H.*(THE_Theta_D.*cos(THE_Psi)+THE_Phi_D.*cos(THE_Theta).*sin(THE_Psi))+cg_to_mot_L.*(THE_Theta_D.*sin(THE_Psi)-THE_Phi_D.*cos(THE_Psi).*cos(THE_Theta))))./2.0+(cg_to_mot_L.*cos(THE_Psi).*cos(THE_Theta).*(THE_Psi_D-THE_Phi_D.*sin(THE_Theta)))./2.0-(cg_to_mot_H.*cos(THE_Theta).*sin(THE_Psi).*(THE_Psi_D-THE_Phi_D.*sin(THE_Theta)))./2.0)-THE_Theta_D.*mprop.*cos(THE_Theta).*(cg_to_mot_H.*cos(THE_Psi)-cg_to_mot_L.*sin(THE_Psi)).*(THE_Z_D.*(-1.0./2.0)+(sin(THE_Theta).*(cg_to_mot_H.*(THE_Theta_D.*cos(THE_Psi)+THE_Phi_D.*cos(THE_Theta).*sin(THE_Psi))-cg_to_mot_L.*(THE_Theta_D.*sin(THE_Psi)-THE_Phi_D.*cos(THE_Psi).*cos(THE_Theta))))./2.0+(cg_to_mot_L.*cos(THE_Psi).*cos(THE_Theta).*(THE_Psi_D-THE_Phi_D.*sin(THE_Theta)))./2.0+(cg_to_mot_H.*cos(THE_Theta).*sin(THE_Psi).*(THE_Psi_D-THE_Phi_D.*sin(THE_Theta)))./2.0)-Tbz_2.*cos(THE_Psi).*cos(THE_Theta).*sin(THE_Theta).*(cg_to_mot_H.*cos(THE_Psi)+cg_to_mot_L.*sin(THE_Psi))-Tbz_4.*cos(THE_Psi).*cos(THE_Theta).*sin(THE_Theta).*(cg_to_mot_H.*cos(THE_Psi)-cg_to_mot_L.*sin(THE_Psi))-(mprop.*cos(THE_Phi).*cos(THE_Theta).*(THE_Psi_D.*cg_to_mot_L.*cos(THE_Psi)-THE_Psi_D.*cg_to_mot_H.*sin(THE_Psi)).*(THE_X_D+cos(THE_Phi).*cos(THE_Theta).*(cg_to_mot_H.*(THE_Theta_D.*cos(THE_Psi)+THE_Phi_D.*cos(THE_Theta).*sin(THE_Psi))+cg_to_mot_L.*(THE_Theta_D.*sin(THE_Psi)-THE_Phi_D.*cos(THE_Psi).*cos(THE_Theta)))+cg_to_mot_H.*(THE_Psi_D-THE_Phi_D.*sin(THE_Theta)).*(cos(THE_Psi).*sin(THE_Phi)-cos(THE_Phi).*sin(THE_Psi).*sin(THE_Theta))+cg_to_mot_L.*(THE_Psi_D-THE_Phi_D.*sin(THE_Theta)).*(sin(THE_Phi).*sin(THE_Psi)+cos(THE_Phi).*cos(THE_Psi).*sin(THE_Theta))))./2.0+(mprop.*cos(THE_Phi).*cos(THE_Theta).*(THE_Psi_D.*cg_to_mot_L.*cos(THE_Psi)+THE_Psi_D.*cg_to_mot_H.*sin(THE_Psi)).*(THE_X_D+cos(THE_Phi).*cos(THE_Theta).*(cg_to_mot_H.*(THE_Theta_D.*cos(THE_Psi)+THE_Phi_D.*cos(THE_Theta).*sin(THE_Psi))-cg_to_mot_L.*(THE_Theta_D.*sin(THE_Psi)-THE_Phi_D.*cos(THE_Psi).*cos(THE_Theta)))+cg_to_mot_H.*(THE_Psi_D-THE_Phi_D.*sin(THE_Theta)).*(cos(THE_Psi).*sin(THE_Phi)-cos(THE_Phi).*sin(THE_Psi).*sin(THE_Theta))-cg_to_mot_L.*(THE_Psi_D-THE_Phi_D.*sin(THE_Theta)).*(sin(THE_Phi).*sin(THE_Psi)+cos(THE_Phi).*cos(THE_Psi).*sin(THE_Theta))))./2.0+Tbz_2.*cos(THE_Phi).*cos(THE_Theta).*(cg_to_mot_H.*cos(THE_Psi)+cg_to_mot_L.*sin(THE_Psi)).*(sin(THE_Phi).*sin(THE_Psi)+cos(THE_Phi).*cos(THE_Psi).*sin(THE_Theta))+Tbz_4.*cos(THE_Phi).*cos(THE_Theta).*(cg_to_mot_H.*cos(THE_Psi)-cg_to_mot_L.*sin(THE_Psi)).*(sin(THE_Phi).*sin(THE_Psi)+cos(THE_Phi).*cos(THE_Psi).*sin(THE_Theta))+(mprop.*cos(THE_Phi).*cos(THE_Theta).*(cg_to_mot_H.*cos(THE_Psi)+cg_to_mot_L.*sin(THE_Psi)).*(cos(THE_Phi).*cos(THE_Theta).*(cg_to_mot_H.*(THE_Psi_D.*THE_Theta_D.*sin(THE_Psi)-THE_Phi_D.*THE_Psi_D.*cos(THE_Psi).*cos(THE_Theta)+THE_Phi_D.*THE_Theta_D.*sin(THE_Psi).*sin(THE_Theta))-cg_to_mot_L.*(THE_Psi_D.*THE_Theta_D.*cos(THE_Psi)+THE_Phi_D.*THE_Psi_D.*cos(THE_Theta).*sin(THE_Psi)+THE_Phi_D.*THE_Theta_D.*cos(THE_Psi).*sin(THE_Theta)))-cg_to_mot_L.*(THE_Psi_D-THE_Phi_D.*sin(THE_Theta)).*(THE_Phi_D.*cos(THE_Phi).*sin(THE_Psi)+THE_Psi_D.*cos(THE_Psi).*sin(THE_Phi)+THE_Theta_D.*cos(THE_Phi).*cos(THE_Psi).*cos(THE_Theta)-THE_Phi_D.*cos(THE_Psi).*sin(THE_Phi).*sin(THE_Theta)-THE_Psi_D.*cos(THE_Phi).*sin(THE_Psi).*sin(THE_Theta))+cg_to_mot_H.*(THE_Psi_D-THE_Phi_D.*sin(THE_Theta)).*(-THE_Phi_D.*cos(THE_Phi).*cos(THE_Psi)+THE_Psi_D.*sin(THE_Phi).*sin(THE_Psi)-THE_Phi_D.*sin(THE_Phi).*sin(THE_Psi).*sin(THE_Theta)+THE_Psi_D.*cos(THE_Phi).*cos(THE_Psi).*sin(THE_Theta)+THE_Theta_D.*cos(THE_Phi).*cos(THE_Theta).*sin(THE_Psi))+THE_Phi_D.*cos(THE_Theta).*sin(THE_Phi).*(cg_to_mot_H.*(THE_Theta_D.*cos(THE_Psi)+THE_Phi_D.*cos(THE_Theta).*sin(THE_Psi))+cg_to_mot_L.*(THE_Theta_D.*sin(THE_Psi)-THE_Phi_D.*cos(THE_Psi).*cos(THE_Theta)))+THE_Theta_D.*cos(THE_Phi).*sin(THE_Theta).*(cg_to_mot_H.*(THE_Theta_D.*cos(THE_Psi)+THE_Phi_D.*cos(THE_Theta).*sin(THE_Psi))+cg_to_mot_L.*(THE_Theta_D.*sin(THE_Psi)-THE_Phi_D.*cos(THE_Psi).*cos(THE_Theta)))+THE_Phi_D.*THE_Theta_D.*cg_to_mot_H.*cos(THE_Theta).*(cos(THE_Psi).*sin(THE_Phi)-cos(THE_Phi).*sin(THE_Psi).*sin(THE_Theta))+THE_Phi_D.*THE_Theta_D.*cg_to_mot_L.*cos(THE_Theta).*(sin(THE_Phi).*sin(THE_Psi)+cos(THE_Phi).*cos(THE_Psi).*sin(THE_Theta))))./2.0+(mprop.*cos(THE_Phi).*cos(THE_Theta).*(cg_to_mot_H.*cos(THE_Psi)-cg_to_mot_L.*sin(THE_Psi)).*(cos(THE_Phi).*cos(THE_Theta).*(cg_to_mot_H.*(THE_Psi_D.*THE_Theta_D.*sin(THE_Psi)-THE_Phi_D.*THE_Psi_D.*cos(THE_Psi).*cos(THE_Theta)+THE_Phi_D.*THE_Theta_D.*sin(THE_Psi).*sin(THE_Theta))+cg_to_mot_L.*(THE_Psi_D.*THE_Theta_D.*cos(THE_Psi)+THE_Phi_D.*THE_Psi_D.*cos(THE_Theta).*sin(THE_Psi)+THE_Phi_D.*THE_Theta_D.*cos(THE_Psi).*sin(THE_Theta)))+cg_to_mot_L.*(THE_Psi_D-THE_Phi_D.*sin(THE_Theta)).*(THE_Phi_D.*cos(THE_Phi).*sin(THE_Psi)+THE_Psi_D.*cos(THE_Psi).*sin(THE_Phi)+THE_Theta_D.*cos(THE_Phi).*cos(THE_Psi).*cos(THE_Theta)-THE_Phi_D.*cos(THE_Psi).*sin(THE_Phi).*sin(THE_Theta)-THE_Psi_D.*cos(THE_Phi).*sin(THE_Psi).*sin(THE_Theta))+cg_to_mot_H.*(THE_Psi_D-THE_Phi_D.*sin(THE_Theta)).*(-THE_Phi_D.*cos(THE_Phi).*cos(THE_Psi)+THE_Psi_D.*sin(THE_Phi).*sin(THE_Psi)-THE_Phi_D.*sin(THE_Phi).*sin(THE_Psi).*sin(THE_Theta)+THE_Psi_D.*cos(THE_Phi).*cos(THE_Psi).*sin(THE_Theta)+THE_Theta_D.*cos(THE_Phi).*cos(THE_Theta).*sin(THE_Psi))+THE_Phi_D.*cos(THE_Theta).*sin(THE_Phi).*(cg_to_mot_H.*(THE_Theta_D.*cos(THE_Psi)+THE_Phi_D.*cos(THE_Theta).*sin(THE_Psi))-cg_to_mot_L.*(THE_Theta_D.*sin(THE_Psi)-THE_Phi_D.*cos(THE_Psi).*cos(THE_Theta)))+THE_Theta_D.*cos(THE_Phi).*sin(THE_Theta).*(cg_to_mot_H.*(THE_Theta_D.*cos(THE_Psi)+THE_Phi_D.*cos(THE_Theta).*sin(THE_Psi))-cg_to_mot_L.*(THE_Theta_D.*sin(THE_Psi)-THE_Phi_D.*cos(THE_Psi).*cos(THE_Theta)))+THE_Phi_D.*THE_Theta_D.*cg_to_mot_H.*cos(THE_Theta).*(cos(THE_Psi).*sin(THE_Phi)-cos(THE_Phi).*sin(THE_Psi).*sin(THE_Theta))-THE_Phi_D.*THE_Theta_D.*cg_to_mot_L.*cos(THE_Theta).*(sin(THE_Phi).*sin(THE_Psi)+cos(THE_Phi).*cos(THE_Psi).*sin(THE_Theta))))./2.0+mprop.*cos(THE_Phi).*cos(THE_Theta).*(cg_to_mot_H.*cos(THE_Psi)+cg_to_mot_L.*sin(THE_Psi)).*((cos(THE_Phi).*cos(THE_Theta).*(cg_to_mot_H.*(THE_Psi_D.*THE_Theta_D.*sin(THE_Psi)-THE_Phi_D.*THE_Psi_D.*cos(THE_Psi).*cos(THE_Theta)+THE_Phi_D.*THE_Theta_D.*sin(THE_Psi).*sin(THE_Theta))-cg_to_mot_L.*(THE_Psi_D.*THE_Theta_D.*cos(THE_Psi)+THE_Phi_D.*THE_Psi_D.*cos(THE_Theta).*sin(THE_Psi)+THE_Phi_D.*THE_Theta_D.*cos(THE_Psi).*sin(THE_Theta))))./2.0-(cg_to_mot_L.*(THE_Psi_D-THE_Phi_D.*sin(THE_Theta)).*(THE_Phi_D.*cos(THE_Phi).*sin(THE_Psi)+THE_Psi_D.*cos(THE_Psi).*sin(THE_Phi)+THE_Theta_D.*cos(THE_Phi).*cos(THE_Psi).*cos(THE_Theta)-THE_Phi_D.*cos(THE_Psi).*sin(THE_Phi).*sin(THE_Theta)-THE_Psi_D.*cos(THE_Phi).*sin(THE_Psi).*sin(THE_Theta)))./2.0+(cg_to_mot_H.*(THE_Psi_D-THE_Phi_D.*sin(THE_Theta)).*(-THE_Phi_D.*cos(THE_Phi).*cos(THE_Psi)+THE_Psi_D.*sin(THE_Phi).*sin(THE_Psi)-THE_Phi_D.*sin(THE_Phi).*sin(THE_Psi).*sin(THE_Theta)+THE_Psi_D.*cos(THE_Phi).*cos(THE_Psi).*sin(THE_Theta)+THE_Theta_D.*cos(THE_Phi).*cos(THE_Theta).*sin(THE_Psi)))./2.0+(THE_Phi_D.*cos(THE_Theta).*sin(THE_Phi).*(cg_to_mot_H.*(THE_Theta_D.*cos(THE_Psi)+THE_Phi_D.*cos(THE_Theta).*sin(THE_Psi))+cg_to_mot_L.*(THE_Theta_D.*sin(THE_Psi)-THE_Phi_D.*cos(THE_Psi).*cos(THE_Theta))))./2.0+(THE_Theta_D.*cos(THE_Phi).*sin(THE_Theta).*(cg_to_mot_H.*(THE_Theta_D.*cos(THE_Psi)+THE_Phi_D.*cos(THE_Theta).*sin(THE_Psi))+cg_to_mot_L.*(THE_Theta_D.*sin(THE_Psi)-THE_Phi_D.*cos(THE_Psi).*cos(THE_Theta))))./2.0+(THE_Phi_D.*THE_Theta_D.*cg_to_mot_H.*cos(THE_Theta).*(cos(THE_Psi).*sin(THE_Phi)-cos(THE_Phi).*sin(THE_Psi).*sin(THE_Theta)))./2.0+(THE_Phi_D.*THE_Theta_D.*cg_to_mot_L.*cos(THE_Theta).*(sin(THE_Phi).*sin(THE_Psi)+cos(THE_Phi).*cos(THE_Psi).*sin(THE_Theta)))./2.0)+mprop.*cos(THE_Phi).*cos(THE_Theta).*(cg_to_mot_H.*cos(THE_Psi)-cg_to_mot_L.*sin(THE_Psi)).*((cos(THE_Phi).*cos(THE_Theta).*(cg_to_mot_H.*(THE_Psi_D.*THE_Theta_D.*sin(THE_Psi)-THE_Phi_D.*THE_Psi_D.*cos(THE_Psi).*cos(THE_Theta)+THE_Phi_D.*THE_Theta_D.*sin(THE_Psi).*sin(THE_Theta))+cg_to_mot_L.*(THE_Psi_D.*THE_Theta_D.*cos(THE_Psi)+THE_Phi_D.*THE_Psi_D.*cos(THE_Theta).*sin(THE_Psi)+THE_Phi_D.*THE_Theta_D.*cos(THE_Psi).*sin(THE_Theta))))./2.0+(cg_to_mot_L.*(THE_Psi_D-THE_Phi_D.*sin(THE_Theta)).*(THE_Phi_D.*cos(THE_Phi).*sin(THE_Psi)+THE_Psi_D.*cos(THE_Psi).*sin(THE_Phi)+THE_Theta_D.*cos(THE_Phi).*cos(THE_Psi).*cos(THE_Theta)-THE_Phi_D.*cos(THE_Psi).*sin(THE_Phi).*sin(THE_Theta)-THE_Psi_D.*cos(THE_Phi).*sin(THE_Psi).*sin(THE_Theta)))./2.0+(cg_to_mot_H.*(THE_Psi_D-THE_Phi_D.*sin(THE_Theta)).*(-THE_Phi_D.*cos(THE_Phi).*cos(THE_Psi)+THE_Psi_D.*sin(THE_Phi).*sin(THE_Psi)-THE_Phi_D.*sin(THE_Phi).*sin(THE_Psi).*sin(THE_Theta)+THE_Psi_D.*cos(THE_Phi).*cos(THE_Psi).*sin(THE_Theta)+THE_Theta_D.*cos(THE_Phi).*cos(THE_Theta).*sin(THE_Psi)))./2.0+(THE_Phi_D.*cos(THE_Theta).*sin(THE_Phi).*(cg_to_mot_H.*(THE_Theta_D.*cos(THE_Psi)+THE_Phi_D.*cos(THE_Theta).*sin(THE_Psi))-cg_to_mot_L.*(THE_Theta_D.*sin(THE_Psi)-THE_Phi_D.*cos(THE_Psi).*cos(THE_Theta))))./2.0+(THE_Theta_D.*cos(THE_Phi).*sin(THE_Theta).*(cg_to_mot_H.*(THE_Theta_D.*cos(THE_Psi)+THE_Phi_D.*cos(THE_Theta).*sin(THE_Psi))-cg_to_mot_L.*(THE_Theta_D.*sin(THE_Psi)-THE_Phi_D.*cos(THE_Psi).*cos(THE_Theta))))./2.0+(THE_Phi_D.*THE_Theta_D.*cg_to_mot_H.*cos(THE_Theta).*(cos(THE_Psi).*sin(THE_Phi)-cos(THE_Phi).*sin(THE_Psi).*sin(THE_Theta)))./2.0-(THE_Phi_D.*THE_Theta_D.*cg_to_mot_L.*cos(THE_Theta).*(sin(THE_Phi).*sin(THE_Psi)+cos(THE_Phi).*cos(THE_Psi).*sin(THE_Theta)))./2.0)+(mprop.*cos(THE_Theta).*sin(THE_Phi).*(THE_Psi_D.*cg_to_mot_L.*cos(THE_Psi)+THE_Psi_D.*cg_to_mot_H.*sin(THE_Psi)).*(THE_Y_D+cos(THE_Theta).*sin(THE_Phi).*(cg_to_mot_H.*(THE_Theta_D.*cos(THE_Psi)+THE_Phi_D.*cos(THE_Theta).*sin(THE_Psi))-cg_to_mot_L.*(THE_Theta_D.*sin(THE_Psi)-THE_Phi_D.*cos(THE_Psi).*cos(THE_Theta)))-cg_to_mot_H.*(THE_Psi_D-THE_Phi_D.*sin(THE_Theta)).*(cos(THE_Phi).*cos(THE_Psi)+sin(THE_Phi).*sin(THE_Psi).*sin(THE_Theta))+cg_to_mot_L.*(THE_Psi_D-THE_Phi_D.*sin(THE_Theta)).*(cos(THE_Phi).*sin(THE_Psi)-cos(THE_Psi).*sin(THE_Phi).*sin(THE_Theta))))./2.0-(mprop.*cos(THE_Theta).*sin(THE_Phi).*(THE_Psi_D.*cg_to_mot_L.*cos(THE_Psi)-THE_Psi_D.*cg_to_mot_H.*sin(THE_Psi)).*(THE_Y_D+cos(THE_Theta).*sin(THE_Phi).*(cg_to_mot_H.*(THE_Theta_D.*cos(THE_Psi)+THE_Phi_D.*cos(THE_Theta).*sin(THE_Psi))+cg_to_mot_L.*(THE_Theta_D.*sin(THE_Psi)-THE_Phi_D.*cos(THE_Psi).*cos(THE_Theta)))-cg_to_mot_H.*(THE_Psi_D-THE_Phi_D.*sin(THE_Theta)).*(cos(THE_Phi).*cos(THE_Psi)+sin(THE_Phi).*sin(THE_Psi).*sin(THE_Theta))-cg_to_mot_L.*(THE_Psi_D-THE_Phi_D.*sin(THE_Theta)).*(cos(THE_Phi).*sin(THE_Psi)-cos(THE_Psi).*sin(THE_Phi).*sin(THE_Theta))))./2.0-Tbz_2.*cos(THE_Theta).*sin(THE_Phi).*(cg_to_mot_H.*cos(THE_Psi)+cg_to_mot_L.*sin(THE_Psi)).*(cos(THE_Phi).*sin(THE_Psi)-cos(THE_Psi).*sin(THE_Phi).*sin(THE_Theta))-Tbz_4.*cos(THE_Theta).*sin(THE_Phi).*(cg_to_mot_H.*cos(THE_Psi)-cg_to_mot_L.*sin(THE_Psi)).*(cos(THE_Phi).*sin(THE_Psi)-cos(THE_Psi).*sin(THE_Phi).*sin(THE_Theta))-(mprop.*cos(THE_Theta).*sin(THE_Phi).*(cg_to_mot_H.*cos(THE_Psi)+cg_to_mot_L.*sin(THE_Psi)).*(-cos(THE_Theta).*sin(THE_Phi).*(cg_to_mot_H.*(THE_Psi_D.*THE_Theta_D.*sin(THE_Psi)-THE_Phi_D.*THE_Psi_D.*cos(THE_Psi).*cos(THE_Theta)+THE_Phi_D.*THE_Theta_D.*sin(THE_Psi).*sin(THE_Theta))-cg_to_mot_L.*(THE_Psi_D.*THE_Theta_D.*cos(THE_Psi)+THE_Phi_D.*THE_Psi_D.*cos(THE_Theta).*sin(THE_Psi)+THE_Phi_D.*THE_Theta_D.*cos(THE_Psi).*sin(THE_Theta)))+cg_to_mot_L.*(THE_Psi_D-THE_Phi_D.*sin(THE_Theta)).*(-THE_Psi_D.*cos(THE_Phi).*cos(THE_Psi)+THE_Phi_D.*sin(THE_Phi).*sin(THE_Psi)-THE_Psi_D.*sin(THE_Phi).*sin(THE_Psi).*sin(THE_Theta)+THE_Phi_D.*cos(THE_Phi).*cos(THE_Psi).*sin(THE_Theta)+THE_Theta_D.*cos(THE_Psi).*cos(THE_Theta).*sin(THE_Phi))-cg_to_mot_H.*(THE_Psi_D-THE_Phi_D.*sin(THE_Theta)).*(-THE_Phi_D.*cos(THE_Psi).*sin(THE_Phi)-THE_Psi_D.*cos(THE_Phi).*sin(THE_Psi)+THE_Phi_D.*cos(THE_Phi).*sin(THE_Psi).*sin(THE_Theta)+THE_Psi_D.*cos(THE_Psi).*sin(THE_Phi).*sin(THE_Theta)+THE_Theta_D.*cos(THE_Theta).*sin(THE_Phi).*sin(THE_Psi))+THE_Phi_D.*cos(THE_Phi).*cos(THE_Theta).*(cg_to_mot_H.*(THE_Theta_D.*cos(THE_Psi)+THE_Phi_D.*cos(THE_Theta).*sin(THE_Psi))+cg_to_mot_L.*(THE_Theta_D.*sin(THE_Psi)-THE_Phi_D.*cos(THE_Psi).*cos(THE_Theta)))-THE_Theta_D.*sin(THE_Phi).*sin(THE_Theta).*(cg_to_mot_H.*(THE_Theta_D.*cos(THE_Psi)+THE_Phi_D.*cos(THE_Theta).*sin(THE_Psi))+cg_to_mot_L.*(THE_Theta_D.*sin(THE_Psi)-THE_Phi_D.*cos(THE_Psi).*cos(THE_Theta)))+THE_Phi_D.*THE_Theta_D.*cg_to_mot_H.*cos(THE_Theta).*(cos(THE_Phi).*cos(THE_Psi)+sin(THE_Phi).*sin(THE_Psi).*sin(THE_Theta))+THE_Phi_D.*THE_Theta_D.*cg_to_mot_L.*cos(THE_Theta).*(cos(THE_Phi).*sin(THE_Psi)-cos(THE_Psi).*sin(THE_Phi).*sin(THE_Theta))))./2.0+(mprop.*cos(THE_Theta).*sin(THE_Phi).*(cg_to_mot_H.*cos(THE_Psi)-cg_to_mot_L.*sin(THE_Psi)).*(cos(THE_Theta).*sin(THE_Phi).*(cg_to_mot_H.*(THE_Psi_D.*THE_Theta_D.*sin(THE_Psi)-THE_Phi_D.*THE_Psi_D.*cos(THE_Psi).*cos(THE_Theta)+THE_Phi_D.*THE_Theta_D.*sin(THE_Psi).*sin(THE_Theta))+cg_to_mot_L.*(THE_Psi_D.*THE_Theta_D.*cos(THE_Psi)+THE_Phi_D.*THE_Psi_D.*cos(THE_Theta).*sin(THE_Psi)+THE_Phi_D.*THE_Theta_D.*cos(THE_Psi).*sin(THE_Theta)))+cg_to_mot_L.*(THE_Psi_D-THE_Phi_D.*sin(THE_Theta)).*(-THE_Psi_D.*cos(THE_Phi).*cos(THE_Psi)+THE_Phi_D.*sin(THE_Phi).*sin(THE_Psi)-THE_Psi_D.*sin(THE_Phi).*sin(THE_Psi).*sin(THE_Theta)+THE_Phi_D.*cos(THE_Phi).*cos(THE_Psi).*sin(THE_Theta)+THE_Theta_D.*cos(THE_Psi).*cos(THE_Theta).*sin(THE_Phi))+cg_to_mot_H.*(THE_Psi_D-THE_Phi_D.*sin(THE_Theta)).*(-THE_Phi_D.*cos(THE_Psi).*sin(THE_Phi)-THE_Psi_D.*cos(THE_Phi).*sin(THE_Psi)+THE_Phi_D.*cos(THE_Phi).*sin(THE_Psi).*sin(THE_Theta)+THE_Psi_D.*cos(THE_Psi).*sin(THE_Phi).*sin(THE_Theta)+THE_Theta_D.*cos(THE_Theta).*sin(THE_Phi).*sin(THE_Psi))-THE_Phi_D.*cos(THE_Phi).*cos(THE_Theta).*(cg_to_mot_H.*(THE_Theta_D.*cos(THE_Psi)+THE_Phi_D.*cos(THE_Theta).*sin(THE_Psi))-cg_to_mot_L.*(THE_Theta_D.*sin(THE_Psi)-THE_Phi_D.*cos(THE_Psi).*cos(THE_Theta)))+THE_Theta_D.*sin(THE_Phi).*sin(THE_Theta).*(cg_to_mot_H.*(THE_Theta_D.*cos(THE_Psi)+THE_Phi_D.*cos(THE_Theta).*sin(THE_Psi))-cg_to_mot_L.*(THE_Theta_D.*sin(THE_Psi)-THE_Phi_D.*cos(THE_Psi).*cos(THE_Theta)))-THE_Phi_D.*THE_Theta_D.*cg_to_mot_H.*cos(THE_Theta).*(cos(THE_Phi).*cos(THE_Psi)+sin(THE_Phi).*sin(THE_Psi).*sin(THE_Theta))+THE_Phi_D.*THE_Theta_D.*cg_to_mot_L.*cos(THE_Theta).*(cos(THE_Phi).*sin(THE_Psi)-cos(THE_Psi).*sin(THE_Phi).*sin(THE_Theta))))./2.0-mprop.*cos(THE_Theta).*sin(THE_Phi).*(cg_to_mot_H.*cos(THE_Psi)+cg_to_mot_L.*sin(THE_Psi)).*(cos(THE_Theta).*sin(THE_Phi).*(cg_to_mot_H.*(THE_Psi_D.*THE_Theta_D.*sin(THE_Psi)-THE_Phi_D.*THE_Psi_D.*cos(THE_Psi).*cos(THE_Theta)+THE_Phi_D.*THE_Theta_D.*sin(THE_Psi).*sin(THE_Theta))-cg_to_mot_L.*(THE_Psi_D.*THE_Theta_D.*cos(THE_Psi)+THE_Phi_D.*THE_Psi_D.*cos(THE_Theta).*sin(THE_Psi)+THE_Phi_D.*THE_Theta_D.*cos(THE_Psi).*sin(THE_Theta))).*(-1.0./2.0)+(cg_to_mot_L.*(THE_Psi_D-THE_Phi_D.*sin(THE_Theta)).*(-THE_Psi_D.*cos(THE_Phi).*cos(THE_Psi)+THE_Phi_D.*sin(THE_Phi).*sin(THE_Psi)-THE_Psi_D.*sin(THE_Phi).*sin(THE_Psi).*sin(THE_Theta)+THE_Phi_D.*cos(THE_Phi).*cos(THE_Psi).*sin(THE_Theta)+THE_Theta_D.*cos(THE_Psi).*cos(THE_Theta).*sin(THE_Phi)))./2.0-(cg_to_mot_H.*(THE_Psi_D-THE_Phi_D.*sin(THE_Theta)).*(-THE_Phi_D.*cos(THE_Psi).*sin(THE_Phi)-THE_Psi_D.*cos(THE_Phi).*sin(THE_Psi)+THE_Phi_D.*cos(THE_Phi).*sin(THE_Psi).*sin(THE_Theta)+THE_Psi_D.*cos(THE_Psi).*sin(THE_Phi).*sin(THE_Theta)+THE_Theta_D.*cos(THE_Theta).*sin(THE_Phi).*sin(THE_Psi)))./2.0+(THE_Phi_D.*cos(THE_Phi).*cos(THE_Theta).*(cg_to_mot_H.*(THE_Theta_D.*cos(THE_Psi)+THE_Phi_D.*cos(THE_Theta).*sin(THE_Psi))+cg_to_mot_L.*(THE_Theta_D.*sin(THE_Psi)-THE_Phi_D.*cos(THE_Psi).*cos(THE_Theta))))./2.0-(THE_Theta_D.*sin(THE_Phi).*sin(THE_Theta).*(cg_to_mot_H.*(THE_Theta_D.*cos(THE_Psi)+THE_Phi_D.*cos(THE_Theta).*sin(THE_Psi))+cg_to_mot_L.*(THE_Theta_D.*sin(THE_Psi)-THE_Phi_D.*cos(THE_Psi).*cos(THE_Theta))))./2.0+(THE_Phi_D.*THE_Theta_D.*cg_to_mot_H.*cos(THE_Theta).*(cos(THE_Phi).*cos(THE_Psi)+sin(THE_Phi).*sin(THE_Psi).*sin(THE_Theta)))./2.0+(THE_Phi_D.*THE_Theta_D.*cg_to_mot_L.*cos(THE_Theta).*(cos(THE_Phi).*sin(THE_Psi)-cos(THE_Psi).*sin(THE_Phi).*sin(THE_Theta)))./2.0)+mprop.*cos(THE_Theta).*sin(THE_Phi).*(cg_to_mot_H.*cos(THE_Psi)-cg_to_mot_L.*sin(THE_Psi)).*((cos(THE_Theta).*sin(THE_Phi).*(cg_to_mot_H.*(THE_Psi_D.*THE_Theta_D.*sin(THE_Psi)-THE_Phi_D.*THE_Psi_D.*cos(THE_Psi).*cos(THE_Theta)+THE_Phi_D.*THE_Theta_D.*sin(THE_Psi).*sin(THE_Theta))+cg_to_mot_L.*(THE_Psi_D.*THE_Theta_D.*cos(THE_Psi)+THE_Phi_D.*THE_Psi_D.*cos(THE_Theta).*sin(THE_Psi)+THE_Phi_D.*THE_Theta_D.*cos(THE_Psi).*sin(THE_Theta))))./2.0+(cg_to_mot_L.*(THE_Psi_D-THE_Phi_D.*sin(THE_Theta)).*(-THE_Psi_D.*cos(THE_Phi).*cos(THE_Psi)+THE_Phi_D.*sin(THE_Phi).*sin(THE_Psi)-THE_Psi_D.*sin(THE_Phi).*sin(THE_Psi).*sin(THE_Theta)+THE_Phi_D.*cos(THE_Phi).*cos(THE_Psi).*sin(THE_Theta)+THE_Theta_D.*cos(THE_Psi).*cos(THE_Theta).*sin(THE_Phi)))./2.0+(cg_to_mot_H.*(THE_Psi_D-THE_Phi_D.*sin(THE_Theta)).*(-THE_Phi_D.*cos(THE_Psi).*sin(THE_Phi)-THE_Psi_D.*cos(THE_Phi).*sin(THE_Psi)+THE_Phi_D.*cos(THE_Phi).*sin(THE_Psi).*sin(THE_Theta)+THE_Psi_D.*cos(THE_Psi).*sin(THE_Phi).*sin(THE_Theta)+THE_Theta_D.*cos(THE_Theta).*sin(THE_Phi).*sin(THE_Psi)))./2.0-(THE_Phi_D.*cos(THE_Phi).*cos(THE_Theta).*(cg_to_mot_H.*(THE_Theta_D.*cos(THE_Psi)+THE_Phi_D.*cos(THE_Theta).*sin(THE_Psi))-cg_to_mot_L.*(THE_Theta_D.*sin(THE_Psi)-THE_Phi_D.*cos(THE_Psi).*cos(THE_Theta))))./2.0+(THE_Theta_D.*sin(THE_Phi).*sin(THE_Theta).*(cg_to_mot_H.*(THE_Theta_D.*cos(THE_Psi)+THE_Phi_D.*cos(THE_Theta).*sin(THE_Psi))-cg_to_mot_L.*(THE_Theta_D.*sin(THE_Psi)-THE_Phi_D.*cos(THE_Psi).*cos(THE_Theta))))./2.0-(THE_Phi_D.*THE_Theta_D.*cg_to_mot_H.*cos(THE_Theta).*(cos(THE_Phi).*cos(THE_Psi)+sin(THE_Phi).*sin(THE_Psi).*sin(THE_Theta)))./2.0+(THE_Phi_D.*THE_Theta_D.*cg_to_mot_L.*cos(THE_Theta).*(cos(THE_Phi).*sin(THE_Psi)-cos(THE_Psi).*sin(THE_Phi).*sin(THE_Theta)))./2.0)+mprop.*cos(THE_Phi).*cos(THE_Theta).*(THE_Psi_D.*cg_to_mot_L.*cos(THE_Psi)+THE_Psi_D.*cg_to_mot_H.*sin(THE_Psi)).*(THE_X_D./2.0+(cos(THE_Phi).*cos(THE_Theta).*(cg_to_mot_H.*(THE_Theta_D.*cos(THE_Psi)+THE_Phi_D.*cos(THE_Theta).*sin(THE_Psi))-cg_to_mot_L.*(THE_Theta_D.*sin(THE_Psi)-THE_Phi_D.*cos(THE_Psi).*cos(THE_Theta))))./2.0+(cg_to_mot_H.*(THE_Psi_D-THE_Phi_D.*sin(THE_Theta)).*(cos(THE_Psi).*sin(THE_Phi)-cos(THE_Phi).*sin(THE_Psi).*sin(THE_Theta)))./2.0-(cg_to_mot_L.*(THE_Psi_D-THE_Phi_D.*sin(THE_Theta)).*(sin(THE_Phi).*sin(THE_Psi)+cos(THE_Phi).*cos(THE_Psi).*sin(THE_Theta)))./2.0)-mprop.*cos(THE_Phi).*cos(THE_Theta).*(THE_Psi_D.*cg_to_mot_L.*cos(THE_Psi)-THE_Psi_D.*cg_to_mot_H.*sin(THE_Psi)).*(THE_X_D./2.0+(cos(THE_Phi).*cos(THE_Theta).*(cg_to_mot_H.*(THE_Theta_D.*cos(THE_Psi)+THE_Phi_D.*cos(THE_Theta).*sin(THE_Psi))+cg_to_mot_L.*(THE_Theta_D.*sin(THE_Psi)-THE_Phi_D.*cos(THE_Psi).*cos(THE_Theta))))./2.0+(cg_to_mot_H.*(THE_Psi_D-THE_Phi_D.*sin(THE_Theta)).*(cos(THE_Psi).*sin(THE_Phi)-cos(THE_Phi).*sin(THE_Psi).*sin(THE_Theta)))./2.0+(cg_to_mot_L.*(THE_Psi_D-THE_Phi_D.*sin(THE_Theta)).*(sin(THE_Phi).*sin(THE_Psi)+cos(THE_Phi).*cos(THE_Psi).*sin(THE_Theta)))./2.0)+(THE_Theta_D.*mprop.*cos(THE_Theta).*(cg_to_mot_H.*cos(THE_Psi)+cg_to_mot_L.*sin(THE_Psi)).*(THE_Z_D-sin(THE_Theta).*(cg_to_mot_H.*(THE_Theta_D.*cos(THE_Psi)+THE_Phi_D.*cos(THE_Theta).*sin(THE_Psi))+cg_to_mot_L.*(THE_Theta_D.*sin(THE_Psi)-THE_Phi_D.*cos(THE_Psi).*cos(THE_Theta)))+cg_to_mot_L.*cos(THE_Psi).*cos(THE_Theta).*(THE_Psi_D-THE_Phi_D.*sin(THE_Theta))-cg_to_mot_H.*cos(THE_Theta).*sin(THE_Psi).*(THE_Psi_D-THE_Phi_D.*sin(THE_Theta))))./2.0+mprop.*cos(THE_Theta).*sin(THE_Phi).*(THE_Psi_D.*cg_to_mot_L.*cos(THE_Psi)+THE_Psi_D.*cg_to_mot_H.*sin(THE_Psi)).*(THE_Y_D./2.0+(cos(THE_Theta).*sin(THE_Phi).*(cg_to_mot_H.*(THE_Theta_D.*cos(THE_Psi)+THE_Phi_D.*cos(THE_Theta).*sin(THE_Psi))-cg_to_mot_L.*(THE_Theta_D.*sin(THE_Psi)-THE_Phi_D.*cos(THE_Psi).*cos(THE_Theta))))./2.0-(cg_to_mot_H.*(THE_Psi_D-THE_Phi_D.*sin(THE_Theta)).*(cos(THE_Phi).*cos(THE_Psi)+sin(THE_Phi).*sin(THE_Psi).*sin(THE_Theta)))./2.0+(cg_to_mot_L.*(THE_Psi_D-THE_Phi_D.*sin(THE_Theta)).*(cos(THE_Phi).*sin(THE_Psi)-cos(THE_Psi).*sin(THE_Phi).*sin(THE_Theta)))./2.0)-mprop.*cos(THE_Theta).*sin(THE_Phi).*(THE_Psi_D.*cg_to_mot_L.*cos(THE_Psi)-THE_Psi_D.*cg_to_mot_H.*sin(THE_Psi)).*(THE_Y_D./2.0+(cos(THE_Theta).*sin(THE_Phi).*(cg_to_mot_H.*(THE_Theta_D.*cos(THE_Psi)+THE_Phi_D.*cos(THE_Theta).*sin(THE_Psi))+cg_to_mot_L.*(THE_Theta_D.*sin(THE_Psi)-THE_Phi_D.*cos(THE_Psi).*cos(THE_Theta))))./2.0-(cg_to_mot_H.*(THE_Psi_D-THE_Phi_D.*sin(THE_Theta)).*(cos(THE_Phi).*cos(THE_Psi)+sin(THE_Phi).*sin(THE_Psi).*sin(THE_Theta)))./2.0-(cg_to_mot_L.*(THE_Psi_D-THE_Phi_D.*sin(THE_Theta)).*(cos(THE_Phi).*sin(THE_Psi)-cos(THE_Psi).*sin(THE_Phi).*sin(THE_Theta)))./2.0)+(THE_Phi_D.*mprop.*cos(THE_Theta).*sin(THE_Phi).*(cg_to_mot_H.*cos(THE_Psi)+cg_to_mot_L.*sin(THE_Psi)).*(THE_X_D+cos(THE_Phi).*cos(THE_Theta).*(cg_to_mot_H.*(THE_Theta_D.*cos(THE_Psi)+THE_Phi_D.*cos(THE_Theta).*sin(THE_Psi))+cg_to_mot_L.*(THE_Theta_D.*sin(THE_Psi)-THE_Phi_D.*cos(THE_Psi).*cos(THE_Theta)))+cg_to_mot_H.*(THE_Psi_D-THE_Phi_D.*sin(THE_Theta)).*(cos(THE_Psi).*sin(THE_Phi)-cos(THE_Phi).*sin(THE_Psi).*sin(THE_Theta))+cg_to_mot_L.*(THE_Psi_D-THE_Phi_D.*sin(THE_Theta)).*(sin(THE_Phi).*sin(THE_Psi)+cos(THE_Phi).*cos(THE_Psi).*sin(THE_Theta))))./2.0-(THE_Phi_D.*mprop.*cos(THE_Phi).*cos(THE_Theta).*(cg_to_mot_H.*cos(THE_Psi)+cg_to_mot_L.*sin(THE_Psi)).*(THE_Y_D+cos(THE_Theta).*sin(THE_Phi).*(cg_to_mot_H.*(THE_Theta_D.*cos(THE_Psi)+THE_Phi_D.*cos(THE_Theta).*sin(THE_Psi))+cg_to_mot_L.*(THE_Theta_D.*sin(THE_Psi)-THE_Phi_D.*cos(THE_Psi).*cos(THE_Theta)))-cg_to_mot_H.*(THE_Psi_D-THE_Phi_D.*sin(THE_Theta)).*(cos(THE_Phi).*cos(THE_Psi)+sin(THE_Phi).*sin(THE_Psi).*sin(THE_Theta))-cg_to_mot_L.*(THE_Psi_D-THE_Phi_D.*sin(THE_Theta)).*(cos(THE_Phi).*sin(THE_Psi)-cos(THE_Psi).*sin(THE_Phi).*sin(THE_Theta))))./2.0+(THE_Phi_D.*mprop.*cos(THE_Theta).*sin(THE_Phi).*(cg_to_mot_H.*cos(THE_Psi)-cg_to_mot_L.*sin(THE_Psi)).*(THE_X_D+cos(THE_Phi).*cos(THE_Theta).*(cg_to_mot_H.*(THE_Theta_D.*cos(THE_Psi)+THE_Phi_D.*cos(THE_Theta).*sin(THE_Psi))-cg_to_mot_L.*(THE_Theta_D.*sin(THE_Psi)-THE_Phi_D.*cos(THE_Psi).*cos(THE_Theta)))+cg_to_mot_H.*(THE_Psi_D-THE_Phi_D.*sin(THE_Theta)).*(cos(THE_Psi).*sin(THE_Phi)-cos(THE_Phi).*sin(THE_Psi).*sin(THE_Theta))-cg_to_mot_L.*(THE_Psi_D-THE_Phi_D.*sin(THE_Theta)).*(sin(THE_Phi).*sin(THE_Psi)+cos(THE_Phi).*cos(THE_Psi).*sin(THE_Theta))))./2.0-(THE_Phi_D.*mprop.*cos(THE_Phi).*cos(THE_Theta).*(cg_to_mot_H.*cos(THE_Psi)-cg_to_mot_L.*sin(THE_Psi)).*(THE_Y_D+cos(THE_Theta).*sin(THE_Phi).*(cg_to_mot_H.*(THE_Theta_D.*cos(THE_Psi)+THE_Phi_D.*cos(THE_Theta).*sin(THE_Psi))-cg_to_mot_L.*(THE_Theta_D.*sin(THE_Psi)-THE_Phi_D.*cos(THE_Psi).*cos(THE_Theta)))-cg_to_mot_H.*(THE_Psi_D-THE_Phi_D.*sin(THE_Theta)).*(cos(THE_Phi).*cos(THE_Psi)+sin(THE_Phi).*sin(THE_Psi).*sin(THE_Theta))+cg_to_mot_L.*(THE_Psi_D-THE_Phi_D.*sin(THE_Theta)).*(cos(THE_Phi).*sin(THE_Psi)-cos(THE_Psi).*sin(THE_Phi).*sin(THE_Theta))))./2.0+(THE_Theta_D.*mprop.*cos(THE_Phi).*sin(THE_Theta).*(cg_to_mot_H.*cos(THE_Psi)+cg_to_mot_L.*sin(THE_Psi)).*(THE_X_D+cos(THE_Phi).*cos(THE_Theta).*(cg_to_mot_H.*(THE_Theta_D.*cos(THE_Psi)+THE_Phi_D.*cos(THE_Theta).*sin(THE_Psi))+cg_to_mot_L.*(THE_Theta_D.*sin(THE_Psi)-THE_Phi_D.*cos(THE_Psi).*cos(THE_Theta)))+cg_to_mot_H.*(THE_Psi_D-THE_Phi_D.*sin(THE_Theta)).*(cos(THE_Psi).*sin(THE_Phi)-cos(THE_Phi).*sin(THE_Psi).*sin(THE_Theta))+cg_to_mot_L.*(THE_Psi_D-THE_Phi_D.*sin(THE_Theta)).*(sin(THE_Phi).*sin(THE_Psi)+cos(THE_Phi).*cos(THE_Psi).*sin(THE_Theta))))./2.0+(THE_Theta_D.*mprop.*cos(THE_Phi).*sin(THE_Theta).*(cg_to_mot_H.*cos(THE_Psi)-cg_to_mot_L.*sin(THE_Psi)).*(THE_X_D+cos(THE_Phi).*cos(THE_Theta).*(cg_to_mot_H.*(THE_Theta_D.*cos(THE_Psi)+THE_Phi_D.*cos(THE_Theta).*sin(THE_Psi))-cg_to_mot_L.*(THE_Theta_D.*sin(THE_Psi)-THE_Phi_D.*cos(THE_Psi).*cos(THE_Theta)))+cg_to_mot_H.*(THE_Psi_D-THE_Phi_D.*sin(THE_Theta)).*(cos(THE_Psi).*sin(THE_Phi)-cos(THE_Phi).*sin(THE_Psi).*sin(THE_Theta))-cg_to_mot_L.*(THE_Psi_D-THE_Phi_D.*sin(THE_Theta)).*(sin(THE_Phi).*sin(THE_Psi)+cos(THE_Phi).*cos(THE_Psi).*sin(THE_Theta))))./2.0+(THE_Theta_D.*mprop.*sin(THE_Phi).*sin(THE_Theta).*(cg_to_mot_H.*cos(THE_Psi)+cg_to_mot_L.*sin(THE_Psi)).*(THE_Y_D+cos(THE_Theta).*sin(THE_Phi).*(cg_to_mot_H.*(THE_Theta_D.*cos(THE_Psi)+THE_Phi_D.*cos(THE_Theta).*sin(THE_Psi))+cg_to_mot_L.*(THE_Theta_D.*sin(THE_Psi)-THE_Phi_D.*cos(THE_Psi).*cos(THE_Theta)))-cg_to_mot_H.*(THE_Psi_D-THE_Phi_D.*sin(THE_Theta)).*(cos(THE_Phi).*cos(THE_Psi)+sin(THE_Phi).*sin(THE_Psi).*sin(THE_Theta))-cg_to_mot_L.*(THE_Psi_D-THE_Phi_D.*sin(THE_Theta)).*(cos(THE_Phi).*sin(THE_Psi)-cos(THE_Psi).*sin(THE_Phi).*sin(THE_Theta))))./2.0+(THE_Theta_D.*mprop.*sin(THE_Phi).*sin(THE_Theta).*(cg_to_mot_H.*cos(THE_Psi)-cg_to_mot_L.*sin(THE_Psi)).*(THE_Y_D+cos(THE_Theta).*sin(THE_Phi).*(cg_to_mot_H.*(THE_Theta_D.*cos(THE_Psi)+THE_Phi_D.*cos(THE_Theta).*sin(THE_Psi))-cg_to_mot_L.*(THE_Theta_D.*sin(THE_Psi)-THE_Phi_D.*cos(THE_Psi).*cos(THE_Theta)))-cg_to_mot_H.*(THE_Psi_D-THE_Phi_D.*sin(THE_Theta)).*(cos(THE_Phi).*cos(THE_Psi)+sin(THE_Phi).*sin(THE_Psi).*sin(THE_Theta))+cg_to_mot_L.*(THE_Psi_D-THE_Phi_D.*sin(THE_Theta)).*(cos(THE_Phi).*sin(THE_Psi)-cos(THE_Psi).*sin(THE_Phi).*sin(THE_Theta))))./2.0+THE_Phi_D.*mprop.*cos(THE_Theta).*sin(THE_Phi).*(cg_to_mot_H.*cos(THE_Psi)+cg_to_mot_L.*sin(THE_Psi)).*(THE_X_D./2.0+(cos(THE_Phi).*cos(THE_Theta).*(cg_to_mot_H.*(THE_Theta_D.*cos(THE_Psi)+THE_Phi_D.*cos(THE_Theta).*sin(THE_Psi))+cg_to_mot_L.*(THE_Theta_D.*sin(THE_Psi)-THE_Phi_D.*cos(THE_Psi).*cos(THE_Theta))))./2.0+(cg_to_mot_H.*(THE_Psi_D-THE_Phi_D.*sin(THE_Theta)).*(cos(THE_Psi).*sin(THE_Phi)-cos(THE_Phi).*sin(THE_Psi).*sin(THE_Theta)))./2.0+(cg_to_mot_L.*(THE_Psi_D-THE_Phi_D.*sin(THE_Theta)).*(sin(THE_Phi).*sin(THE_Psi)+cos(THE_Phi).*cos(THE_Psi).*sin(THE_Theta)))./2.0)-THE_Phi_D.*mprop.*cos(THE_Phi).*cos(THE_Theta).*(cg_to_mot_H.*cos(THE_Psi)+cg_to_mot_L.*sin(THE_Psi)).*(THE_Y_D./2.0+(cos(THE_Theta).*sin(THE_Phi).*(cg_to_mot_H.*(THE_Theta_D.*cos(THE_Psi)+THE_Phi_D.*cos(THE_Theta).*sin(THE_Psi))+cg_to_mot_L.*(THE_Theta_D.*sin(THE_Psi)-THE_Phi_D.*cos(THE_Psi).*cos(THE_Theta))))./2.0-(cg_to_mot_H.*(THE_Psi_D-THE_Phi_D.*sin(THE_Theta)).*(cos(THE_Phi).*cos(THE_Psi)+sin(THE_Phi).*sin(THE_Psi).*sin(THE_Theta)))./2.0-(cg_to_mot_L.*(THE_Psi_D-THE_Phi_D.*sin(THE_Theta)).*(cos(THE_Phi).*sin(THE_Psi)-cos(THE_Psi).*sin(THE_Phi).*sin(THE_Theta)))./2.0)+THE_Phi_D.*mprop.*cos(THE_Theta).*sin(THE_Phi).*(cg_to_mot_H.*cos(THE_Psi)-cg_to_mot_L.*sin(THE_Psi)).*(THE_X_D./2.0+(cos(THE_Phi).*cos(THE_Theta).*(cg_to_mot_H.*(THE_Theta_D.*cos(THE_Psi)+THE_Phi_D.*cos(THE_Theta).*sin(THE_Psi))-cg_to_mot_L.*(THE_Theta_D.*sin(THE_Psi)-THE_Phi_D.*cos(THE_Psi).*cos(THE_Theta))))./2.0+(cg_to_mot_H.*(THE_Psi_D-THE_Phi_D.*sin(THE_Theta)).*(cos(THE_Psi).*sin(THE_Phi)-cos(THE_Phi).*sin(THE_Psi).*sin(THE_Theta)))./2.0-(cg_to_mot_L.*(THE_Psi_D-THE_Phi_D.*sin(THE_Theta)).*(sin(THE_Phi).*sin(THE_Psi)+cos(THE_Phi).*cos(THE_Psi).*sin(THE_Theta)))./2.0)-THE_Phi_D.*mprop.*cos(THE_Phi).*cos(THE_Theta).*(cg_to_mot_H.*cos(THE_Psi)-cg_to_mot_L.*sin(THE_Psi)).*(THE_Y_D./2.0+(cos(THE_Theta).*sin(THE_Phi).*(cg_to_mot_H.*(THE_Theta_D.*cos(THE_Psi)+THE_Phi_D.*cos(THE_Theta).*sin(THE_Psi))-cg_to_mot_L.*(THE_Theta_D.*sin(THE_Psi)-THE_Phi_D.*cos(THE_Psi).*cos(THE_Theta))))./2.0-(cg_to_mot_H.*(THE_Psi_D-THE_Phi_D.*sin(THE_Theta)).*(cos(THE_Phi).*cos(THE_Psi)+sin(THE_Phi).*sin(THE_Psi).*sin(THE_Theta)))./2.0+(cg_to_mot_L.*(THE_Psi_D-THE_Phi_D.*sin(THE_Theta)).*(cos(THE_Phi).*sin(THE_Psi)-cos(THE_Psi).*sin(THE_Phi).*sin(THE_Theta)))./2.0)+THE_Theta_D.*mprop.*cos(THE_Phi).*sin(THE_Theta).*(cg_to_mot_H.*cos(THE_Psi)+cg_to_mot_L.*sin(THE_Psi)).*(THE_X_D./2.0+(cos(THE_Phi).*cos(THE_Theta).*(cg_to_mot_H.*(THE_Theta_D.*cos(THE_Psi)+THE_Phi_D.*cos(THE_Theta).*sin(THE_Psi))+cg_to_mot_L.*(THE_Theta_D.*sin(THE_Psi)-THE_Phi_D.*cos(THE_Psi).*cos(THE_Theta))))./2.0+(cg_to_mot_H.*(THE_Psi_D-THE_Phi_D.*sin(THE_Theta)).*(cos(THE_Psi).*sin(THE_Phi)-cos(THE_Phi).*sin(THE_Psi).*sin(THE_Theta)))./2.0+(cg_to_mot_L.*(THE_Psi_D-THE_Phi_D.*sin(THE_Theta)).*(sin(THE_Phi).*sin(THE_Psi)+cos(THE_Phi).*cos(THE_Psi).*sin(THE_Theta)))./2.0)+THE_Theta_D.*mprop.*cos(THE_Phi).*sin(THE_Theta).*(cg_to_mot_H.*cos(THE_Psi)-cg_to_mot_L.*sin(THE_Psi)).*(THE_X_D./2.0+(cos(THE_Phi).*cos(THE_Theta).*(cg_to_mot_H.*(THE_Theta_D.*cos(THE_Psi)+THE_Phi_D.*cos(THE_Theta).*sin(THE_Psi))-cg_to_mot_L.*(THE_Theta_D.*sin(THE_Psi)-THE_Phi_D.*cos(THE_Psi).*cos(THE_Theta))))./2.0+(cg_to_mot_H.*(THE_Psi_D-THE_Phi_D.*sin(THE_Theta)).*(cos(THE_Psi).*sin(THE_Phi)-cos(THE_Phi).*sin(THE_Psi).*sin(THE_Theta)))./2.0-(cg_to_mot_L.*(THE_Psi_D-THE_Phi_D.*sin(THE_Theta)).*(sin(THE_Phi).*sin(THE_Psi)+cos(THE_Phi).*cos(THE_Psi).*sin(THE_Theta)))./2.0)+THE_Theta_D.*mprop.*sin(THE_Phi).*sin(THE_Theta).*(cg_to_mot_H.*cos(THE_Psi)+cg_to_mot_L.*sin(THE_Psi)).*(THE_Y_D./2.0+(cos(THE_Theta).*sin(THE_Phi).*(cg_to_mot_H.*(THE_Theta_D.*cos(THE_Psi)+THE_Phi_D.*cos(THE_Theta).*sin(THE_Psi))+cg_to_mot_L.*(THE_Theta_D.*sin(THE_Psi)-THE_Phi_D.*cos(THE_Psi).*cos(THE_Theta))))./2.0-(cg_to_mot_H.*(THE_Psi_D-THE_Phi_D.*sin(THE_Theta)).*(cos(THE_Phi).*cos(THE_Psi)+sin(THE_Phi).*sin(THE_Psi).*sin(THE_Theta)))./2.0-(cg_to_mot_L.*(THE_Psi_D-THE_Phi_D.*sin(THE_Theta)).*(cos(THE_Phi).*sin(THE_Psi)-cos(THE_Psi).*sin(THE_Phi).*sin(THE_Theta)))./2.0)+THE_Theta_D.*mprop.*sin(THE_Phi).*sin(THE_Theta).*(cg_to_mot_H.*cos(THE_Psi)-cg_to_mot_L.*sin(THE_Psi)).*(THE_Y_D./2.0+(cos(THE_Theta).*sin(THE_Phi).*(cg_to_mot_H.*(THE_Theta_D.*cos(THE_Psi)+THE_Phi_D.*cos(THE_Theta).*sin(THE_Psi))-cg_to_mot_L.*(THE_Theta_D.*sin(THE_Psi)-THE_Phi_D.*cos(THE_Psi).*cos(THE_Theta))))./2.0-(cg_to_mot_H.*(THE_Psi_D-THE_Phi_D.*sin(THE_Theta)).*(cos(THE_Phi).*cos(THE_Psi)+sin(THE_Phi).*sin(THE_Psi).*sin(THE_Theta)))./2.0+(cg_to_mot_L.*(THE_Psi_D-THE_Phi_D.*sin(THE_Theta)).*(cos(THE_Phi).*sin(THE_Psi)-cos(THE_Psi).*sin(THE_Phi).*sin(THE_Theta)))./2.0);